simulink model "Skematik (Bismillah)"  (R2024b)
settings: Solver=ode23tb  StartTime=0.0  StopTime=10.0  RelTol=1e-3
undefined symbols (not defined in the file): D1, Delta
libraries: spsThreePhaseBreakerLib x78, spsThreePhaseParallelRLCLoadLib x39, spsThreePhasePISectionLineLib x26, spsThreePhaseTransformerTwoWindingsLib x18, spsExcitationSystemLib x4, spsSynchronousMachinepuStandardLib x4, spsMultimeterLib x1, spspowerguiLib x1
settings Model: Creator=Laika  LastModifiedBy=ACER
settings SolverCC: AlgebraicLoopSolver=TrustRegion
settings ModelReferenceCC: EnableRefExpFcnMdlSchedulingChecks=on
settings RTWCC: GPUComputeCapability=3.5  DLArmComputeVersion=19.05

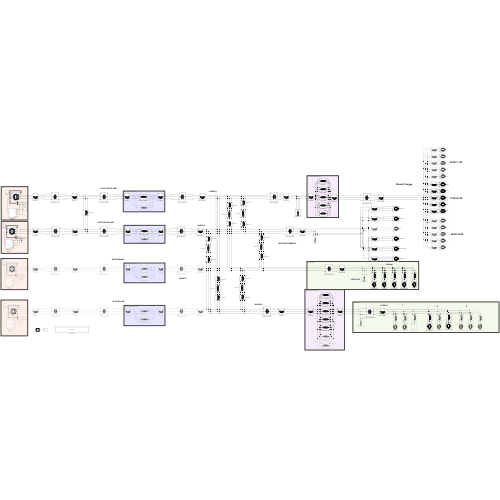
[thumbnail: Simulink's stored preview of the top-level diagram]
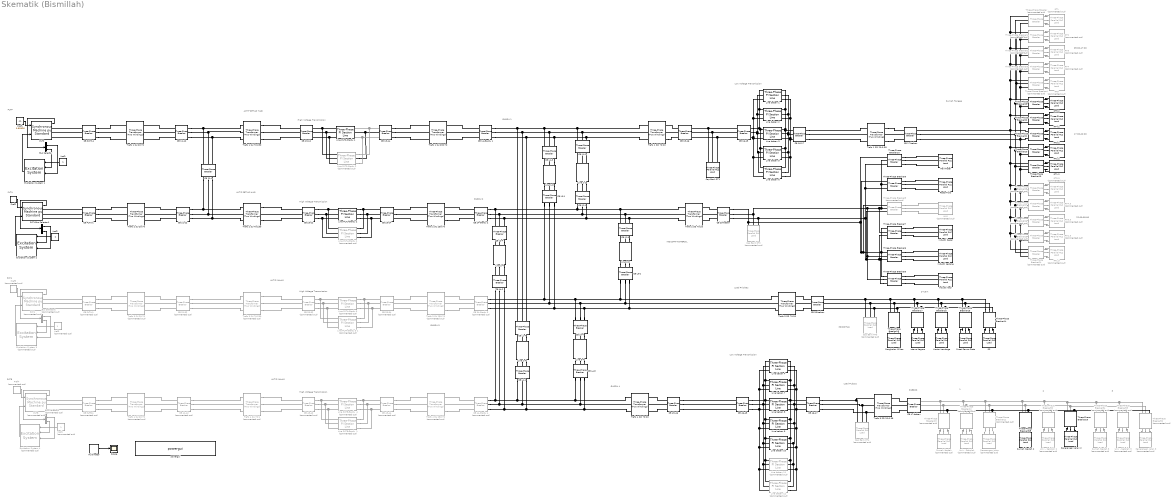
== system Skematik (Bismillah) ==
  note: High Voltage Transmission
  note: High Voltage Transmission
  note: High Voltage Transmission
  note: High Voltage Transmission
  note: Low Voltage Transmission
  note: Load Pubsos
  note: Load Prioritas
  note: Low Voltage Transmission
  note: PLTB
  note: PLTA
  note: PLTU
  note: PLTP
  note: GARDU 2
  note: GARDU 1
  note: GARDU 3
  note: GARDU 4
  note: AKTIF MALAM
  note: AKTIF MALAM
  note: AKTIF SETIAP HARI
  note: AKTIF SETIAP HARI
  note: INDUSTRI-KOMERSIL
  note: PRIORITAS
  note: PUBSOS
  note: 05:00-17:00
  note: 24 Jam
  note: 1
  note: 3
  note: 2
  note: 17:00-22:00
  note: 22:00-05:00
  note: Rumah Tangga
  Bus Selector : BusSelector  OutputSignals="dq0 components.Stator voltage  vq (pu),dq0 components.Stator voltage  vd (pu)"
  Bus Selector1 : BusSelector  OutputSignals="dq0 components.Stator voltage  vq (pu),dq0 components.Stator voltage  vd (pu)"
  Bus Selector2 : BusSelector  Commented=on  OutputSignals="dq0 components.Stator voltage  vq (pu),dq0 components.Stator voltage  vd (pu)"
  Bus Selector3 : BusSelector  Commented=on  OutputSignals="dq0 components.Stator voltage  vq (pu),dq0 components.Stator voltage  vd (pu)"
  CB 11-1 : spsThreePhaseBreakerLib/Three-Phase Breaker  InitialState=closed  SwitchA=off  SwitchB=off  SwitchC=off  SwitchTimes="[4/60  10/60]"  External=off  BreakerResistance=0.001  SnubberResistance=1e6  SnubberCapacitance=inf  Measurements=None
  CB 11-12 : spsThreePhaseBreakerLib/Three-Phase Breaker  InitialState=closed  SwitchA=off  SwitchB=off  SwitchC=off  SwitchTimes="[4/60  10/60]"  External=off  BreakerResistance=0.001  SnubberResistance=1e6  SnubberCapacitance=inf  Measurements=None
  CB 13-12 : spsThreePhaseBreakerLib/Three-Phase Breaker  InitialState=closed  SwitchA=off  SwitchB=off  SwitchC=off  SwitchTimes="[4/60  10/60]"  External=off  BreakerResistance=0.001  SnubberResistance=1e6  SnubberCapacitance=inf  Measurements=None
  CB 13-14 : spsThreePhaseBreakerLib/Three-Phase Breaker  InitialState=closed  SwitchA=off  SwitchB=off  SwitchC=off  SwitchTimes="[4/60  10/60]"  External=off  BreakerResistance=0.001  SnubberResistance=1e6  SnubberCapacitance=inf  Measurements=None
  CB 14-Gardu 1 : spsThreePhaseBreakerLib/Three-Phase Breaker  InitialState=closed  SwitchA=off  SwitchB=off  SwitchC=off  SwitchTimes="[4/60  10/60]"  External=off  BreakerResistance=0.001  SnubberResistance=1e6  SnubberCapacitance=inf  Measurements=None
  CB 15-16 : spsThreePhaseBreakerLib/Three-Phase Breaker  InitialState=closed  SwitchA=off  SwitchB=off  SwitchC=off  SwitchTimes="[4/60  10/60]"  External=off  BreakerResistance=0.001  SnubberResistance=1e6  SnubberCapacitance=inf  Measurements=None
  CB 16-15 : spsThreePhaseBreakerLib/Three-Phase Breaker  InitialState=closed  SwitchA=off  SwitchB=off  SwitchC=off  SwitchTimes="[4/60  10/60]"  External=off  BreakerResistance=0.001  SnubberResistance=1e6  SnubberCapacitance=inf  Measurements=None
  CB 16-17 : spsThreePhaseBreakerLib/Three-Phase Breaker  InitialState=closed  SwitchA=off  SwitchB=off  SwitchC=off  SwitchTimes="[4/60  10/60]"  External=off  BreakerResistance=0.001  SnubberResistance=1e6  SnubberCapacitance=inf  Measurements=None
  CB 17-beban : spsThreePhaseBreakerLib/Three-Phase Breaker  InitialState=closed  SwitchA=off  SwitchB=off  SwitchC=off  SwitchTimes="[4/60  10/60]"  External=off  BreakerResistance=1e-7  SnubberResistance=1e6  SnubberCapacitance=inf  Measurements=None
  CB 21-22 : spsThreePhaseBreakerLib/Three-Phase Breaker  InitialState=closed  SwitchA=off  SwitchB=off  SwitchC=off  SwitchTimes="[4/60  10/60]"  External=off  BreakerResistance=0.001  SnubberResistance=1e6  SnubberCapacitance=inf  Measurements=None
  CB 23-22 : spsThreePhaseBreakerLib/Three-Phase Breaker  InitialState=closed  SwitchA=off  SwitchB=off  SwitchC=off  SwitchTimes="[4/60  10/60]"  External=off  BreakerResistance=0.001  SnubberResistance=1e6  SnubberCapacitance=inf  Measurements=None
  CB 23-24 : spsThreePhaseBreakerLib/Three-Phase Breaker  InitialState=closed  SwitchA=off  SwitchB=off  SwitchC=off  SwitchTimes="[4/60  10/60]"  External=off  BreakerResistance=0.001  SnubberResistance=1e6  SnubberCapacitance=inf  Measurements=None
  CB 24-Gardu 2 : spsThreePhaseBreakerLib/Three-Phase Breaker  InitialState=closed  SwitchA=off  SwitchB=off  SwitchC=off  SwitchTimes="[4/60  10/60]"  External=off  BreakerResistance=0.001  SnubberResistance=1e6  SnubberCapacitance=inf  Measurements=None
  CB 25-beban : spsThreePhaseBreakerLib/Three-Phase Breaker  InitialState=closed  SwitchA=off  SwitchB=off  SwitchC=off  SwitchTimes="[4/60  10/60]"  External=off  BreakerResistance=1e-7  SnubberResistance=1e6  SnubberCapacitance=inf  Measurements=None
  CB 31-32 : spsThreePhaseBreakerLib/Three-Phase Breaker  Commented=on  InitialState=closed  SwitchA=off  SwitchB=off  SwitchC=off  SwitchTimes="[4/60  10/60]"  External=off  BreakerResistance=0.001  SnubberResistance=1e6  SnubberCapacitance=inf  Measurements=None
  CB 33-32 : spsThreePhaseBreakerLib/Three-Phase Breaker  Commented=on  InitialState=closed  SwitchA=off  SwitchB=off  SwitchC=off  SwitchTimes="[4/60  10/60]"  External=off  BreakerResistance=0.001  SnubberResistance=1e6  SnubberCapacitance=inf  Measurements=None
  CB 33-34 : spsThreePhaseBreakerLib/Three-Phase Breaker  Commented=on  InitialState=closed  SwitchA=off  SwitchB=off  SwitchC=off  SwitchTimes="[4/60  10/60]"  External=off  BreakerResistance=0.001  SnubberResistance=1e6  SnubberCapacitance=inf  Measurements=None
  CB 34-Gardu 3 : spsThreePhaseBreakerLib/Three-Phase Breaker  Commented=on  InitialState=closed  SwitchA=off  SwitchB=off  SwitchC=off  SwitchTimes="[4/60  10/60]"  External=off  BreakerResistance=0.001  SnubberResistance=1e6  SnubberCapacitance=inf  Measurements=None
  CB 35-beban : spsThreePhaseBreakerLib/Three-Phase Breaker  InitialState=closed  SwitchA=off  SwitchB=off  SwitchC=off  SwitchTimes="[4/60  10/60]"  External=off  BreakerResistance=1e-7  SnubberResistance=1e6  SnubberCapacitance=inf  Measurements=None
  CB 41-42 : spsThreePhaseBreakerLib/Three-Phase Breaker  Commented=on  InitialState=closed  SwitchA=off  SwitchB=off  SwitchC=off  SwitchTimes="[4/60  10/60]"  External=off  BreakerResistance=0.001  SnubberResistance=1e6  SnubberCapacitance=inf  Measurements=None
  CB 43-42 : spsThreePhaseBreakerLib/Three-Phase Breaker  Commented=on  InitialState=closed  SwitchA=off  SwitchB=off  SwitchC=off  SwitchTimes="[4/60  10/60]"  External=off  BreakerResistance=0.001  SnubberResistance=1e6  SnubberCapacitance=inf  Measurements=None
  CB 43-44 : spsThreePhaseBreakerLib/Three-Phase Breaker  Commented=on  InitialState=closed  SwitchA=off  SwitchB=off  SwitchC=off  SwitchTimes="[4/60  10/60]"  External=off  BreakerResistance=0.001  SnubberResistance=1e6  SnubberCapacitance=inf  Measurements=None
  CB 44-Gardu 4 : spsThreePhaseBreakerLib/Three-Phase Breaker  Commented=on  InitialState=closed  SwitchA=off  SwitchB=off  SwitchC=off  SwitchTimes="[4/60  10/60]"  External=off  BreakerResistance=0.001  SnubberResistance=1e6  SnubberCapacitance=inf  Measurements=None
  CB 45-46 : spsThreePhaseBreakerLib/Three-Phase Breaker  InitialState=closed  SwitchA=off  SwitchB=off  SwitchC=off  SwitchTimes="[4/60  10/60]"  External=off  BreakerResistance=0.001  SnubberResistance=1e6  SnubberCapacitance=inf  Measurements=None
  CB 46-45 : spsThreePhaseBreakerLib/Three-Phase Breaker  InitialState=closed  SwitchA=off  SwitchB=off  SwitchC=off  SwitchTimes="[4/60  10/60]"  External=off  BreakerResistance=0.001  SnubberResistance=1e6  SnubberCapacitance=inf  Measurements=None
  CB 46-47 : spsThreePhaseBreakerLib/Three-Phase Breaker  InitialState=closed  SwitchA=off  SwitchB=off  SwitchC=off  SwitchTimes="[4/60  10/60]"  External=off  BreakerResistance=0.001  SnubberResistance=1e6  SnubberCapacitance=inf  Measurements=None
  CB 47-beban : spsThreePhaseBreakerLib/Three-Phase Breaker  InitialState=closed  SwitchA=off  SwitchB=off  SwitchC=off  SwitchTimes="[4/60  10/60]"  External=off  BreakerResistance=1e-7  SnubberResistance=1e6  SnubberCapacitance=inf  Measurements=None
  CB L1-2 : spsThreePhaseBreakerLib/Three-Phase Breaker  InitialState=closed  SwitchA=off  SwitchB=off  SwitchC=off  SwitchTimes="[4/60  10/60]"  External=off  BreakerResistance=0.001  SnubberResistance=1e6  SnubberCapacitance=inf  Measurements=None
  CB L1-3 : spsThreePhaseBreakerLib/Three-Phase Breaker  InitialState=closed  SwitchA=off  SwitchB=off  SwitchC=off  SwitchTimes="[4/60  10/60]"  External=off  BreakerResistance=0.001  SnubberResistance=1e6  SnubberCapacitance=inf  Measurements=None
  CB L1-4 : spsThreePhaseBreakerLib/Three-Phase Breaker  InitialState=closed  SwitchA=off  SwitchB=off  SwitchC=off  SwitchTimes="[4/60  10/60]"  External=off  BreakerResistance=0.001  SnubberResistance=1e6  SnubberCapacitance=inf  Measurements=None
  CB L2-1 : spsThreePhaseBreakerLib/Three-Phase Breaker  InitialState=closed  SwitchA=off  SwitchB=off  SwitchC=off  SwitchTimes="[4/60  10/60]"  External=off  BreakerResistance=0.001  SnubberResistance=1e6  SnubberCapacitance=inf  Measurements=None
  CB L2-3 : spsThreePhaseBreakerLib/Three-Phase Breaker  InitialState=closed  SwitchA=off  SwitchB=off  SwitchC=off  SwitchTimes="[4/60  10/60]"  External=off  BreakerResistance=0.001  SnubberResistance=1e6  SnubberCapacitance=inf  Measurements=None
  CB L2-4 : spsThreePhaseBreakerLib/Three-Phase Breaker  InitialState=closed  SwitchA=off  SwitchB=off  SwitchC=off  SwitchTimes="[4/60  10/60]"  External=off  BreakerResistance=0.001  SnubberResistance=1e6  SnubberCapacitance=inf  Measurements=None
  CB L3-1 : spsThreePhaseBreakerLib/Three-Phase Breaker  InitialState=closed  SwitchA=off  SwitchB=off  SwitchC=off  SwitchTimes="[4/60  10/60]"  External=off  BreakerResistance=0.001  SnubberResistance=1e6  SnubberCapacitance=inf  Measurements=None
  CB L3-2 : spsThreePhaseBreakerLib/Three-Phase Breaker  InitialState=closed  SwitchA=off  SwitchB=off  SwitchC=off  SwitchTimes="[4/60  10/60]"  External=off  BreakerResistance=0.001  SnubberResistance=1e6  SnubberCapacitance=inf  Measurements=None
  CB L3-4 : spsThreePhaseBreakerLib/Three-Phase Breaker  InitialState=closed  SwitchA=off  SwitchB=off  SwitchC=off  SwitchTimes="[4/60  10/60]"  External=off  BreakerResistance=0.001  SnubberResistance=1e6  SnubberCapacitance=inf  Measurements=None
  CB L4-1 : spsThreePhaseBreakerLib/Three-Phase Breaker  InitialState=closed  SwitchA=off  SwitchB=off  SwitchC=off  SwitchTimes="[4/60  10/60]"  External=off  BreakerResistance=0.001  SnubberResistance=1e6  SnubberCapacitance=inf  Measurements=None
  CB L4-2 : spsThreePhaseBreakerLib/Three-Phase Breaker  InitialState=closed  SwitchA=off  SwitchB=off  SwitchC=off  SwitchTimes="[4/60  10/60]"  External=off  BreakerResistance=0.001  SnubberResistance=1e6  SnubberCapacitance=inf  Measurements=None
  CB L4-3 : spsThreePhaseBreakerLib/Three-Phase Breaker  InitialState=closed  SwitchA=off  SwitchB=off  SwitchC=off  SwitchTimes="[4/60  10/60]"  External=off  BreakerResistance=0.001  SnubberResistance=1e6  SnubberCapacitance=inf  Measurements=None
  CB PLTA-1 : spsThreePhaseBreakerLib/Three-Phase Breaker  Commented=on  InitialState=closed  SwitchA=off  SwitchB=off  SwitchC=off  SwitchTimes="[4/60  10/60]"  External=off  BreakerResistance=0.001  SnubberResistance=1e6  SnubberCapacitance=inf  Measurements=None
  CB PLTB-1 : spsThreePhaseBreakerLib/Three-Phase Breaker  Commented=on  InitialState=closed  SwitchA=off  SwitchB=off  SwitchC=off  SwitchTimes="[4/60  10/60]"  External=off  BreakerResistance=0.001  SnubberResistance=1e6  SnubberCapacitance=inf  Measurements=None
  CB PLTP-1 : spsThreePhaseBreakerLib/Three-Phase Breaker  InitialState=closed  SwitchA=off  SwitchB=off  SwitchC=off  SwitchTimes="[4/60  10/60]"  External=off  BreakerResistance=0.001  SnubberResistance=1e6  SnubberCapacitance=inf  Measurements=None
  CB PLTU-1 : spsThreePhaseBreakerLib/Three-Phase Breaker  InitialState=closed  SwitchA=off  SwitchB=off  SwitchC=off  SwitchTimes="[4/60  10/60]"  External=off  BreakerResistance=0.001  SnubberResistance=1e6  SnubberCapacitance=inf  Measurements=None
  Cap Bank RT1 : spsThreePhaseParallelRLCLoadLib/Three-Phase Parallel RLC Load  LConnTagsString=A|B|C  Configuration=Y (grounded)  NominalVoltage=20e3  Vabc=[1e3 1e3 1e3]  Vabcp=[1e3 1e3 1e3]  NominalFrequency=50  UnbalancedPower=off  ActivePower=0  InductivePower=0  CapacitivePower=60e6  Pabc=[10e3 9e3 11e3]  QLabc=[100 90 110]  QCabc=[100 90 110]  Pabcp=[10e3 9e3 11e3]  QLabcp=[100 90 110]  QCabcp=[100 90 110]  Measurements=Branch voltages and currents  LoadType=constant Z
  Cap Bank RT2 : spsThreePhaseParallelRLCLoadLib/Three-Phase Parallel RLC Load  Commented=on  LConnTagsString=A|B|C  Configuration=Y (grounded)  NominalVoltage=20e3  Vabc=[1e3 1e3 1e3]  Vabcp=[1e3 1e3 1e3]  NominalFrequency=50  UnbalancedPower=off  ActivePower=0  InductivePower=0  CapacitivePower=50e3  Pabc=[10e3 9e3 11e3]  QLabc=[100 90 110]  QCabc=[100 90 110]  Pabcp=[10e3 9e3 11e3]  QLabcp=[100 90 110]  QCabcp=[100 90 110]  Measurements=Branch voltages and currents  LoadType=constant Z
  Cap Bank RT3 : spsThreePhaseParallelRLCLoadLib/Three-Phase Parallel RLC Load  Commented=on  LConnTagsString=A|B|C  Configuration=Y (grounded)  NominalVoltage=20e3  Vabc=[1e3 1e3 1e3]  Vabcp=[1e3 1e3 1e3]  NominalFrequency=50  UnbalancedPower=off  ActivePower=0  InductivePower=0  CapacitivePower=50e3  Pabc=[10e3 9e3 11e3]  QLabc=[100 90 110]  QCabc=[100 90 110]  Pabcp=[10e3 9e3 11e3]  QLabcp=[100 90 110]  QCabcp=[100 90 110]  Measurements=Branch voltages and currents  LoadType=constant Z
  Cap Bank RT4 : spsThreePhaseParallelRLCLoadLib/Three-Phase Parallel RLC Load  Commented=on  LConnTagsString=A|B|C  Configuration=Y (grounded)  NominalVoltage=20e3  Vabc=[1e3 1e3 1e3]  Vabcp=[1e3 1e3 1e3]  NominalFrequency=50  UnbalancedPower=off  ActivePower=0  InductivePower=0  CapacitivePower=0.75e6  Pabc=[10e3 9e3 11e3]  QLabc=[100 90 110]  QCabc=[100 90 110]  Pabcp=[10e3 9e3 11e3]  QLabcp=[100 90 110]  QCabcp=[100 90 110]  Measurements=Branch voltages and currents  LoadType=constant Z
  Excitation System 1 : spsExcitationSystemLib/Excitation System  tr=20e-3  reg=[ 300, 0.001 ]  exc=[ 1, 0 ]  tgr=[ 0, 0 ]  damp=[ 0.001, 0.1 ]  sat=[ 0, 0 ]  lim=[ -11.5, 11.5, 0 ]  v0=[1 18.415]
  Excitation System 2 : spsExcitationSystemLib/Excitation System  tr=20e-3  reg=[ 300, 0.001 ]  exc=[ 1, 0 ]  tgr=[ 0, 0 ]  damp=[ 0.001, 0.1 ]  sat=[ 0, 0 ]  lim=[ -11.5, 11.5, 0 ]  v0=[1 13.043]
  Excitation System 3 : spsExcitationSystemLib/Excitation System  Commented=on  tr=20e-3  reg=[ 300, 0.001 ]  exc=[ 1, 0 ]  tgr=[ 0, 0 ]  damp=[ 0.001, 0.1 ]  sat=[ 0, 0 ]  lim=[ -11.5, 11.5, 0 ]  v0=[1 2.1735]
  Excitation System 4 : spsExcitationSystemLib/Excitation System  Commented=on  tr=20e-3  reg=[ 300, 0.001 ]  exc=[ 1, 0 ]  tgr=[ 0, 0 ]  damp=[ 0.001, 0.1 ]  sat=[ 0, 0 ]  lim=[ -11.5, 11.5, 0 ]  v0=[1 12.474]
  Industri besar : spsThreePhaseParallelRLCLoadLib/Three-Phase Parallel RLC Load  LConnTagsString=A|B|C  Configuration=Y (grounded)  NominalVoltage=20e3  Vabc=[1e3 1e3 1e3]  Vabcp=[1e3 1e3 1e3]  NominalFrequency=50  UnbalancedPower=off  ActivePower=9e5  InductivePower=4.36e5  CapacitivePower=0  Pabc=[10e3 9e3 11e3]  QLabc=[100 90 110]  QCabc=[100 90 110]  Pabcp=[10e3 9e3 11e3]  QLabcp=[100 90 110]  QCabcp=[100 90 110]  Measurements=Branch voltages and currents  LoadType=constant Z
  Industri kecil : spsThreePhaseParallelRLCLoadLib/Three-Phase Parallel RLC Load  LConnTagsString=A|B|C  Configuration=Y (grounded)  NominalVoltage=20e3  Vabc=[1e3 1e3 1e3]  Vabcp=[1e3 1e3 1e3]  NominalFrequency=50  UnbalancedPower=off  ActivePower=5.94e5  InductivePower=2.88e5  CapacitivePower=0  Pabc=[10e3 9e3 11e3]  QLabc=[100 90 110]  QCabc=[100 90 110]  Pabcp=[10e3 9e3 11e3]  QLabcp=[100 90 110]  QCabcp=[100 90 110]  Measurements=Branch voltages and currents  LoadType=constant Z
  Industri sedang : spsThreePhaseParallelRLCLoadLib/Three-Phase Parallel RLC Load  LConnTagsString=A|B|C  Configuration=Y (grounded)  NominalVoltage=20e3  Vabc=[1e3 1e3 1e3]  Vabcp=[1e3 1e3 1e3]  NominalFrequency=50  UnbalancedPower=off  ActivePower=4.5e6  InductivePower=2.18e6  CapacitivePower=0  Pabc=[10e3 9e3 11e3]  QLabc=[100 90 110]  QCabc=[100 90 110]  Pabcp=[10e3 9e3 11e3]  QLabcp=[100 90 110]  QCabcp=[100 90 110]  Measurements=Branch voltages and currents  LoadType=constant Z
  Istana Negara : spsThreePhaseParallelRLCLoadLib/Three-Phase Parallel RLC Load  LConnTagsString=A|B|C  Configuration=Y (grounded)  NominalVoltage=20e3  Vabc=[1e3 1e3 1e3]  Vabcp=[1e3 1e3 1e3]  NominalFrequency=50  UnbalancedPower=off  ActivePower=9e4  InductivePower=4.36e4  CapacitivePower=0  Pabc=[10e3 9e3 11e3]  QLabc=[100 90 110]  QCabc=[100 90 110]  Pabcp=[10e3 9e3 11e3]  QLabcp=[100 90 110]  QCabcp=[100 90 110]  Measurements=Branch voltages and currents  LoadType=constant Z
  Kantor Lembaga : spsThreePhaseParallelRLCLoadLib/Three-Phase Parallel RLC Load  LConnTagsString=A|B|C  Configuration=Y (grounded)  NominalVoltage=20e3  Vabc=[1e3 1e3 1e3]  Vabcp=[1e3 1e3 1e3]  NominalFrequency=50  UnbalancedPower=off  ActivePower=9e4  InductivePower=4.36e4  CapacitivePower=0  Pabc=[10e3 9e3 11e3]  QLabc=[100 90 110]  QCabc=[100 90 110]  Pabcp=[10e3 9e3 11e3]  QLabcp=[100 90 110]  QCabcp=[100 90 110]  Measurements=Branch voltages and currents  LoadType=constant Z
  Line 1-1 : spsThreePhasePISectionLineLib/Three-Phase PI Section Line  LConnTagsString=a|b|c  RConnTagsString=A|B|C  Length=20  Frequency=50  Resistances=[ 0.002 0.3864]  Inductances="[ 6.3694e-3  4.1264e-3]"  Capacitances=[12.74e-9 7.751e-9]
  Line 1-3 : spsThreePhasePISectionLineLib/Three-Phase PI Section Line  LConnTagsString=a|b|c  RConnTagsString=A|B|C  Length=5  Frequency=50  Resistances=[ 0.002 0.3864]  Inductances="[ 6.3694e-3  4.1264e-3]"  Capacitances=[12.74e-9 7.751e-9]
  Line 1-4 : spsThreePhasePISectionLineLib/Three-Phase PI Section Line  LConnTagsString=a|b|c  RConnTagsString=A|B|C  Length=20  Frequency=50  Resistances=[ 0.002 0.3864]  Inductances="[ 6.3694e-3  4.1264e-3]"  Capacitances=[12.74e-9 7.751e-9]
  Line 2-3 : spsThreePhasePISectionLineLib/Three-Phase PI Section Line  LConnTagsString=a|b|c  RConnTagsString=A|B|C  Length=5  Frequency=50  Resistances=[ 0.002 0.3864]  Inductances="[ 6.3694e-3  4.1264e-3]"  Capacitances=[12.74e-9 7.751e-9]
  Line 2-4 : spsThreePhasePISectionLineLib/Three-Phase PI Section Line  LConnTagsString=a|b|c  RConnTagsString=A|B|C  Length=20  Frequency=50  Resistances=[ 0.002 0.3864]  Inductances="[ 6.3694e-3  4.1264e-3]"  Capacitances=[12.74e-9 7.751e-9]
  Line 3-4 : spsThreePhasePISectionLineLib/Three-Phase PI Section Line  LConnTagsString=a|b|c  RConnTagsString=A|B|C  Length=5  Frequency=50  Resistances=[ 0.002 0.3864]  Inductances="[ 6.3694e-3  4.1264e-3]"  Capacitances=[12.74e-9 7.751e-9]
  "Line PLTA-Gardu 3 " : spsThreePhasePISectionLineLib/Three-Phase PI Section Line  Commented=on  LConnTagsString=a|b|c  RConnTagsString=A|B|C  Length=50  Frequency=50  Resistances=[ 0.002 0.3864]  Inductances="[ 6.3694e-3  4.1264e-3]"  Capacitances=[12.74e-9 7.751e-9]
  Line PLTA-Gardu 3 1 : spsThreePhasePISectionLineLib/Three-Phase PI Section Line  Commented=on  LConnTagsString=a|b|c  RConnTagsString=A|B|C  Length=50  Frequency=50  Resistances=[ 0.002 0.3864]  Inductances="[ 6.3694e-3  4.1264e-3]"  Capacitances=[12.74e-9 7.751e-9]
  Line PLTB-Gardu  1 : spsThreePhasePISectionLineLib/Three-Phase PI Section Line  Commented=on  LConnTagsString=a|b|c  RConnTagsString=A|B|C  Length=20  Frequency=50  Resistances=[ 0.002 0.3864]  Inductances="[ 6.3694e-3  4.1264e-3]"  Capacitances=[12.74e-9 7.751e-9]
  Line PLTB-Gardu  4 : spsThreePhasePISectionLineLib/Three-Phase PI Section Line  Commented=on  LConnTagsString=a|b|c  RConnTagsString=A|B|C  Length=20  Frequency=50  Resistances=[ 0.002 0.3864]  Inductances="[ 6.3694e-3  4.1264e-3]"  Capacitances=[12.74e-9 7.751e-9]
  Line PLTP-Gardu 1 : spsThreePhasePISectionLineLib/Three-Phase PI Section Line  LConnTagsString=a|b|c  RConnTagsString=A|B|C  Length=100  Frequency=50  Resistances=[ 0.002 0.3864]  Inductances="[ 6.3694e-3  4.1264e-3]"  Capacitances=[12.74e-9 7.751e-9]
  Line PLTP-Gardu 2 : spsThreePhasePISectionLineLib/Three-Phase PI Section Line  Commented=on  LConnTagsString=a|b|c  RConnTagsString=A|B|C  Length=100  Frequency=50  Resistances=[ 0.002 0.3864]  Inductances="[ 6.3694e-3  4.1264e-3]"  Capacitances=[12.74e-9 7.751e-9]
  Line PLTU-Gardu 1 : spsThreePhasePISectionLineLib/Three-Phase PI Section Line  Commented=on  LConnTagsString=a|b|c  RConnTagsString=A|B|C  Length=100  Frequency=50  Resistances=[ 0.002 0.3864]  Inductances="[ 6.3694e-3  4.1264e-3]"  Capacitances=[12.74e-9 7.751e-9]
  Line PLTU-Gardu 2 : spsThreePhasePISectionLineLib/Three-Phase PI Section Line  LConnTagsString=a|b|c  RConnTagsString=A|B|C  Length=100  Frequency=50  Resistances=[ 0.002 0.3864]  Inductances="[ 6.3694e-3  4.1264e-3]"  Capacitances=[12.74e-9 7.751e-9]
  Line beban {1..10} (10 alike) : spsThreePhasePISectionLineLib/Three-Phase PI Section Line  LConnTagsString=a|b|c  RConnTagsString=A|B|C  Length=3  Frequency=50  Resistances=[ 0.002 0.3864]  Inductances="[ 6.3694e-3  4.1264e-3]"  Capacitances=[12.74e-9 7.751e-9]
  Line beban 11 : spsThreePhasePISectionLineLib/Three-Phase PI Section Line  Commented=on  LConnTagsString=a|b|c  RConnTagsString=A|B|C  Length=3  Frequency=50  Resistances=[ 0.002 0.3864]  Inductances="[ 6.3694e-3  4.1264e-3]"  Capacitances=[12.74e-9 7.751e-9]
  Line beban 12 : spsThreePhasePISectionLineLib/Three-Phase PI Section Line  Commented=on  LConnTagsString=a|b|c  RConnTagsString=A|B|C  Length=3  Frequency=50  Resistances=[ 0.002 0.3864]  Inductances="[ 6.3694e-3  4.1264e-3]"  Capacitances=[12.74e-9 7.751e-9]
  Mall-Hotel : spsThreePhaseParallelRLCLoadLib/Three-Phase Parallel RLC Load  LConnTagsString=A|B|C  Configuration=Y (grounded)  NominalVoltage=20e3  Vabc=[1e3 1e3 1e3]  Vabcp=[1e3 1e3 1e3]  NominalFrequency=50  UnbalancedPower=off  ActivePower=9e4  InductivePower=4.36e4  CapacitivePower=0  Pabc=[10e3 9e3 11e3]  QLabc=[100 90 110]  QCabc=[100 90 110]  Pabcp=[10e3 9e3 11e3]  QLabcp=[100 90 110]  QCabcp=[100 90 110]  Measurements=Branch voltages and currents  LoadType=constant Z
  Multimeter : spsMultimeterLib/Multimeter  L=216  sel=[7 8 9 10 11 12 13 14 15 16 17 18 19 20 21 22 23 24 25 26 27 34 35 36 37 38 39 67 68 69 76 77 78 85 86 87 97 98 99]  yselected={}  Gain=[1 1 1 1 1 1 1 1 1 1 1 1 1 1 1 1 1 1 1 1 1 1 1 1 1 1 1 1 1 1 1 1 1 1 1 1 1 1 1]  OutputType=Magnitude  PlotAtSimulationStop=off  PhasorSimulation=off
  PLTA : spsSynchronousMachinepuStandardLib/Synchronous Machine pu Standard  Commented=on  PresetModel=No  MechanicalLoad=Mechanical power Pm  ShowDetailedParameters=on  RotorType=Salient-pole  Units=per unit standard parameters  MeasurementBus=off  NominalParameters="[ 30e6/0.95  20e3   50]"  Reactances1=[ 1.81, 0.3, 0.23, 1.76, 0.65, 0.25, 0.15 ]  Reactances2="[ 1.305, 0.296, 0.252, 0.474,  0.243,  0.1 ]"  dAxisTimeConstants=Open-circuit  qAxisTimeConstants=Short-circuit  TimeConstants1="[ 4.4849  0.0681  0.1  ]"  TimeConstants2=[ 8.0, 0.03, 1.0, 0.07 ]  TimeConstants3="[  4.49  0.0681  0.0513  ]"  TimeConstants4=[ 8.0, 0.03, 0.3371, 0.0295 ]  TimeConstants5=[ 1.01, 0.053, 0.1 ]  TimeConstants6=[ 1.3201, 0.023, 1.0, 0.07 ]  TimeConstants7=[0.012 0.003 0.003]  TimeConstants8=[ 1.3201, 0.0231, 0.3371, 0.0295 ]  StatorResistance=0.003  Mechanical=[ 3.7 0 20 ]  PolePairs=20  InitialConditions=[0 -124.504 1.57718 1.57718 1.57718 -173.405 -293.405 -53.4047 2.17353]  SetSaturation=off  Saturation=[0.6404,0.7127,0.8441,0.9214,0.9956,1.082,1.19,1.316,1.457;0.7,0.7698,0.8872,0.9466,0.9969,1.046,1.1,1.151,1.201]  LoadFlowParameters=[1 120000000 0 0 0]  TsPowergui=0  TsBlock=-1  IterativeModel=Forward Euler  IterativeDiscreteModel=Trapezoidal non iterative  BusType=swing  Pref=100000000  Qref=0  Qmin=-Inf  Qmax=Inf  PLF=0  QLF=0
  PLTB : spsSynchronousMachinepuStandardLib/Synchronous Machine pu Standard  Commented=on  PresetModel=No  MechanicalLoad=Mechanical power Pm  ShowDetailedParameters=on  RotorType=Salient-pole  Units=per unit standard parameters  MeasurementBus=off  NominalParameters="[ 10e6/0.96  20e3   50]"  Reactances1=[ 1.81, 0.3, 0.23, 1.76, 0.65, 0.25, 0.15 ]  Reactances2="[ 1.305, 0.296, 0.252, 0.474,  0.243,  0.1 ]"  dAxisTimeConstants=Open-circuit  qAxisTimeConstants=Short-circuit  TimeConstants1="[ 4.4849  0.0681  0.1  ]"  TimeConstants2=[ 8.0, 0.03, 1.0, 0.07 ]  TimeConstants3="[  4.49  0.0681  0.0513  ]"  TimeConstants4=[ 8.0, 0.03, 0.3371, 0.0295 ]  TimeConstants5=[ 1.01, 0.053, 0.1 ]  TimeConstants6=[ 1.3201, 0.023, 1.0, 0.07 ]  TimeConstants7=[0.012 0.003 0.003]  TimeConstants8=[ 1.3201, 0.0231, 0.3371, 0.0295 ]  StatorResistance=0.003  Mechanical=[ 3.7 0 20 ]  PolePairs=20  InitialConditions=[0 -1.70334 9.60252 9.60252 9.60252 10.9686 -109.031 130.969 12.474]  SetSaturation=off  Saturation=[0.6404,0.7127,0.8441,0.9214,0.9956,1.082,1.19,1.316,1.457;0.7,0.7698,0.8872,0.9466,0.9969,1.046,1.1,1.151,1.201]  LoadFlowParameters=[1 120000000 0 0 0]  TsPowergui=0  TsBlock=-1  IterativeModel=Forward Euler  IterativeDiscreteModel=Trapezoidal non iterative  BusType=PV  Pref=100000000  Qref=0  Qmin=-Inf  Qmax=Inf  PLF=0  QLF=0
  PLTP : spsSynchronousMachinepuStandardLib/Synchronous Machine pu Standard  PresetModel=No  MechanicalLoad=Mechanical power Pm  ShowDetailedParameters=on  RotorType=Salient-pole  Units=per unit standard parameters  MeasurementBus=off  NominalParameters="[ 80e6/0.9  20e3   50]"  Reactances1=[ 1.81, 0.3, 0.23, 1.76, 0.65, 0.25, 0.15 ]  Reactances2="[ 1.305, 0.296, 0.252, 0.474,  0.243,  0.1 ]"  dAxisTimeConstants=Open-circuit  qAxisTimeConstants=Short-circuit  TimeConstants1="[ 4.4849  0.0681  0.1  ]"  TimeConstants2=[ 8.0, 0.03, 1.0, 0.07 ]  TimeConstants3="[  4.49  0.0681  0.0513  ]"  TimeConstants4=[ 8.0, 0.03, 0.3371, 0.0295 ]  TimeConstants5=[ 1.01, 0.053, 0.1 ]  TimeConstants6=[ 1.3201, 0.023, 1.0, 0.07 ]  TimeConstants7=[0.012 0.003 0.003]  TimeConstants8=[ 1.3201, 0.0231, 0.3371, 0.0295 ]  StatorResistance=0.003  Mechanical=[ 3.7 0 20 ]  PolePairs=20  InitialConditions=[0 -89.1081 13.3449 13.3449 13.3449 -88.6045 -208.604 31.3955 18.4147]  SetSaturation=off  Saturation=[0.6404,0.7127,0.8441,0.9214,0.9956,1.082,1.19,1.316,1.457;0.7,0.7698,0.8872,0.9466,0.9969,1.046,1.1,1.151,1.201]  LoadFlowParameters=[2 0 0 0 0]  TsPowergui=0  TsBlock=-1  IterativeModel=Forward Euler  IterativeDiscreteModel=Trapezoidal non iterative  BusType=swing  Pref=0  Qref=0  Qmin=-Inf  Qmax=Inf  PLF=0  QLF=0
  PLTU : spsSynchronousMachinepuStandardLib/Synchronous Machine pu Standard  PresetModel=No  MechanicalLoad=Mechanical power Pm  ShowDetailedParameters=on  RotorType=Salient-pole  Units=per unit standard parameters  MeasurementBus=off  NominalParameters="[ 100e6/0.9  20e3   50]"  Reactances1=[ 1.81, 0.3, 0.23, 1.76, 0.65, 0.25, 0.15 ]  Reactances2="[ 1.305, 0.296, 0.252, 0.474,  0.243,  0.1 ]"  dAxisTimeConstants=Open-circuit  qAxisTimeConstants=Short-circuit  TimeConstants1="[ 4.4849  0.0681  0.1  ]"  TimeConstants2=[ 8.0, 0.03, 1.0, 0.07 ]  TimeConstants3="[  4.49  0.0681  0.0513  ]"  TimeConstants4=[ 8.0, 0.03, 0.3371, 0.0295 ]  TimeConstants5=[ 1.01, 0.053, 0.1 ]  TimeConstants6=[ 1.3201, 0.023, 1.0, 0.07 ]  TimeConstants7=[0.012 0.003 0.003]  TimeConstants8=[ 1.3201, 0.0231, 0.3371, 0.0295 ]  StatorResistance=0.003  Mechanical=[ 3.7 0 20 ]  PolePairs=20  InitialConditions=[0 89.4306 10.7601 10.7601 10.7601 91.0487 -28.9513 211.049 13.0435]  SetSaturation=off  Saturation=[0.6404,0.7127,0.8441,0.9214,0.9956,1.082,1.19,1.316,1.457;0.7,0.7698,0.8872,0.9466,0.9969,1.046,1.1,1.151,1.201]  LoadFlowParameters=[1 120000000 0 0 0]  TsPowergui=0  TsBlock=-1  IterativeModel=Forward Euler  IterativeDiscreteModel=Trapezoidal non iterative  BusType=PV  Pref=100000000  Qref=0  Qmin=-Inf  Qmax=Inf  PLF=0  QLF=0
  Pangkalan Militer : spsThreePhaseParallelRLCLoadLib/Three-Phase Parallel RLC Load  LConnTagsString=A|B|C  Configuration=Y (grounded)  NominalVoltage=20e3  Vabc=[1e3 1e3 1e3]  Vabcp=[1e3 1e3 1e3]  NominalFrequency=50  UnbalancedPower=off  ActivePower=2.03e5  InductivePower=9.81e4  CapacitivePower=0  Pabc=[10e3 9e3 11e3]  QLabc=[100 90 110]  QCabc=[100 90 110]  Pabcp=[10e3 9e3 11e3]  QLabcp=[100 90 110]  QCabcp=[100 90 110]  Measurements=Branch voltages and currents  LoadType=constant Z
  Penerangan Jalan : spsThreePhaseParallelRLCLoadLib/Three-Phase Parallel RLC Load  Commented=on  LConnTagsString=A|B|C  Configuration=Y (grounded)  NominalVoltage=380  Vabc=[1e3 1e3 1e3]  Vabcp=[1e3 1e3 1e3]  NominalFrequency=50  UnbalancedPower=off  ActivePower=0  InductivePower=0  CapacitivePower=0  Pabc=[10e3 9e3 11e3]  QLabc=[100 90 110]  QCabc=[100 90 110]  Pabcp=[10e3 9e3 11e3]  QLabcp=[100 90 110]  QCabcp=[100 90 110]  Measurements=Branch voltages and currents  LoadType=constant Z
  Penerangan Jalan 2 : spsThreePhaseParallelRLCLoadLib/Three-Phase Parallel RLC Load  LConnTagsString=A|B|C  Configuration=Y (grounded)  NominalVoltage=380  Vabc=[1e3 1e3 1e3]  Vabcp=[1e3 1e3 1e3]  NominalFrequency=50  UnbalancedPower=off  ActivePower=1.8e5  InductivePower=8.72e4  CapacitivePower=0  Pabc=[10e3 9e3 11e3]  QLabc=[100 90 110]  QCabc=[100 90 110]  Pabcp=[10e3 9e3 11e3]  QLabcp=[100 90 110]  QCabcp=[100 90 110]  Measurements=Branch voltages and currents  LoadType=constant Z
  Penerangan Jalan 3 : spsThreePhaseParallelRLCLoadLib/Three-Phase Parallel RLC Load  Commented=on  LConnTagsString=A|B|C  Configuration=Y (grounded)  NominalVoltage=380  Vabc=[1e3 1e3 1e3]  Vabcp=[1e3 1e3 1e3]  NominalFrequency=50  UnbalancedPower=off  ActivePower=1.92e6  InductivePower=0.56e6  CapacitivePower=0  Pabc=[10e3 9e3 11e3]  QLabc=[100 90 110]  QCabc=[100 90 110]  Pabcp=[10e3 9e3 11e3]  QLabcp=[100 90 110]  QCabcp=[100 90 110]  Measurements=Branch voltages and currents  LoadType=constant Z
  Pref1 : Constant  Value=0.85926
  Pref2 : Constant  Value=1.2473
  Pref3 : Constant  Commented=on  Value=-1.5593
  Pref4 : Constant  Commented=on  Value=9.8766
  Pusat Server Data : spsThreePhaseParallelRLCLoadLib/Three-Phase Parallel RLC Load  LConnTagsString=A|B|C  Configuration=Y (grounded)  NominalVoltage=20e3  Vabc=[1e3 1e3 1e3]  Vabcp=[1e3 1e3 1e3]  NominalFrequency=50  UnbalancedPower=off  ActivePower=2.25e3  InductivePower=1.09e5  CapacitivePower=0  Pabc=[10e3 9e3 11e3]  QLabc=[100 90 110]  QCabc=[100 90 110]  Pabcp=[10e3 9e3 11e3]  QLabcp=[100 90 110]  QCabcp=[100 90 110]  Measurements=Branch voltages and currents  LoadType=constant Z
  RS : spsThreePhaseParallelRLCLoadLib/Three-Phase Parallel RLC Load  LConnTagsString=A|B|C  Configuration=Y (grounded)  NominalVoltage=20e3  Vabc=[1e3 1e3 1e3]  Vabcp=[1e3 1e3 1e3]  NominalFrequency=50  UnbalancedPower=off  ActivePower=9e4  InductivePower=4.36e4  CapacitivePower=0  Pabc=[10e3 9e3 11e3]  QLabc=[100 90 110]  QCabc=[100 90 110]  Pabcp=[10e3 9e3 11e3]  QLabcp=[100 90 110]  QCabcp=[100 90 110]  Measurements=Branch voltages and currents  LoadType=constant Z
  RT1 : spsThreePhaseParallelRLCLoadLib/Three-Phase Parallel RLC Load  Commented=on  LConnTagsString=A|B|C  Configuration=Y (grounded)  NominalVoltage=380  Vabc=[1e3 1e3 1e3]  Vabcp=[1e3 1e3 1e3]  NominalFrequency=50  UnbalancedPower=off  ActivePower=0.88e6  InductivePower=0.389879952e6  CapacitivePower=0  Pabc=[10e3 9e3 11e3]  QLabc=[100 90 110]  QCabc=[100 90 110]  Pabcp=[10e3 9e3 11e3]  QLabcp=[100 90 110]  QCabcp=[100 90 110]  Measurements=Branch voltages and currents  LoadType=constant Z
  RT1.2 : spsThreePhaseParallelRLCLoadLib/Three-Phase Parallel RLC Load  LConnTagsString=A|B|C  Configuration=Y (grounded)  NominalVoltage=380  Vabc=[1e3 1e3 1e3]  Vabcp=[1e3 1e3 1e3]  NominalFrequency=50  UnbalancedPower=off  ActivePower=1.4e6  InductivePower=6.78e5  CapacitivePower=0  Pabc=[10e3 9e3 11e3]  QLabc=[100 90 110]  QCabc=[100 90 110]  Pabcp=[10e3 9e3 11e3]  QLabcp=[100 90 110]  QCabcp=[100 90 110]  Measurements=Branch voltages and currents  LoadType=constant Z
  RT1.3 : spsThreePhaseParallelRLCLoadLib/Three-Phase Parallel RLC Load  Commented=on  LConnTagsString=A|B|C  Configuration=Y (grounded)  NominalVoltage=380  Vabc=[1e3 1e3 1e3]  Vabcp=[1e3 1e3 1e3]  NominalFrequency=50  UnbalancedPower=off  ActivePower=840000  InductivePower=727461.3392  CapacitivePower=0  Pabc=[10e3 9e3 11e3]  QLabc=[100 90 110]  QCabc=[100 90 110]  Pabcp=[10e3 9e3 11e3]  QLabcp=[100 90 110]  QCabcp=[100 90 110]  Measurements=Branch voltages and currents  LoadType=constant Z
  RT2 : spsThreePhaseParallelRLCLoadLib/Three-Phase Parallel RLC Load  Commented=on  LConnTagsString=A|B|C  Configuration=Y (grounded)  NominalVoltage=380  Vabc=[1e3 1e3 1e3]  Vabcp=[1e3 1e3 1e3]  NominalFrequency=50  UnbalancedPower=off  ActivePower=2.8e7  InductivePower=1.36e7  CapacitivePower=0  Pabc=[10e3 9e3 11e3]  QLabc=[100 90 110]  QCabc=[100 90 110]  Pabcp=[10e3 9e3 11e3]  QLabcp=[100 90 110]  QCabcp=[100 90 110]  Measurements=Branch voltages and currents  LoadType=constant Z
  RT2.2 : spsThreePhaseParallelRLCLoadLib/Three-Phase Parallel RLC Load  LConnTagsString=A|B|C  Configuration=Y (grounded)  NominalVoltage=380  Vabc=[1e3 1e3 1e3]  Vabcp=[1e3 1e3 1e3]  NominalFrequency=50  UnbalancedPower=off  ActivePower=2.8e6  InductivePower=1.36e6  CapacitivePower=0  Pabc=[10e3 9e3 11e3]  QLabc=[100 90 110]  QCabc=[100 90 110]  Pabcp=[10e3 9e3 11e3]  QLabcp=[100 90 110]  QCabcp=[100 90 110]  Measurements=Branch voltages and currents  LoadType=constant Z
  RT2.3 : spsThreePhaseParallelRLCLoadLib/Three-Phase Parallel RLC Load  Commented=on  LConnTagsString=A|B|C  Configuration=Y (grounded)  NominalVoltage=380  Vabc=[1e3 1e3 1e3]  Vabcp=[1e3 1e3 1e3]  NominalFrequency=50  UnbalancedPower=off  ActivePower=6000000  InductivePower=4984871.131  CapacitivePower=0  Pabc=[10e3 9e3 11e3]  QLabc=[100 90 110]  QCabc=[100 90 110]  Pabcp=[10e3 9e3 11e3]  QLabcp=[100 90 110]  QCabcp=[100 90 110]  Measurements=Branch voltages and currents  LoadType=constant Z
  RT3 : spsThreePhaseParallelRLCLoadLib/Three-Phase Parallel RLC Load  Commented=on  LConnTagsString=A|B|C  Configuration=Y (grounded)  NominalVoltage=380  Vabc=[1e3 1e3 1e3]  Vabcp=[1e3 1e3 1e3]  NominalFrequency=50  UnbalancedPower=off  ActivePower=1.19e7  InductivePower=5.76e6  CapacitivePower=0  Pabc=[10e3 9e3 11e3]  QLabc=[100 90 110]  QCabc=[100 90 110]  Pabcp=[10e3 9e3 11e3]  QLabcp=[100 90 110]  QCabcp=[100 90 110]  Measurements=Branch voltages and currents  LoadType=constant Z
  RT3.2 : spsThreePhaseParallelRLCLoadLib/Three-Phase Parallel RLC Load  LConnTagsString=A|B|C  Configuration=Y (grounded)  NominalVoltage=380  Vabc=[1e3 1e3 1e3]  Vabcp=[1e3 1e3 1e3]  NominalFrequency=50  UnbalancedPower=off  ActivePower=1.19e6  InductivePower=5.76e6  CapacitivePower=0  Pabc=[10e3 9e3 11e3]  QLabc=[100 90 110]  QCabc=[100 90 110]  Pabcp=[10e3 9e3 11e3]  QLabcp=[100 90 110]  QCabcp=[100 90 110]  Measurements=Branch voltages and currents  LoadType=constant Z
  RT3.3 : spsThreePhaseParallelRLCLoadLib/Three-Phase Parallel RLC Load  Commented=on  LConnTagsString=A|B|C  Configuration=Y (grounded)  NominalVoltage=380  Vabc=[1e3 1e3 1e3]  Vabcp=[1e3 1e3 1e3]  NominalFrequency=50  UnbalancedPower=off  ActivePower=7700000  InductivePower=6483524.479  CapacitivePower=0  Pabc=[10e3 9e3 11e3]  QLabc=[100 90 110]  QCabc=[100 90 110]  Pabcp=[10e3 9e3 11e3]  QLabcp=[100 90 110]  QCabcp=[100 90 110]  Measurements=Branch voltages and currents  LoadType=constant Z
  RT4 : spsThreePhaseParallelRLCLoadLib/Three-Phase Parallel RLC Load  Commented=on  LConnTagsString=A|B|C  Configuration=Y (grounded)  NominalVoltage=380  Vabc=[1e3 1e3 1e3]  Vabcp=[1e3 1e3 1e3]  NominalFrequency=50  UnbalancedPower=off  ActivePower=4.90e6  InductivePower=2.37e6  CapacitivePower=0  Pabc=[10e3 9e3 11e3]  QLabc=[100 90 110]  QCabc=[100 90 110]  Pabcp=[10e3 9e3 11e3]  QLabcp=[100 90 110]  QCabcp=[100 90 110]  Measurements=Branch voltages and currents  LoadType=constant Z
  RT4.2 : spsThreePhaseParallelRLCLoadLib/Three-Phase Parallel RLC Load  LConnTagsString=A|B|C  Configuration=Y (grounded)  NominalVoltage=380  Vabc=[1e3 1e3 1e3]  Vabcp=[1e3 1e3 1e3]  NominalFrequency=50  UnbalancedPower=off  ActivePower=4.9e5  InductivePower=2.37e5  CapacitivePower=0  Pabc=[10e3 9e3 11e3]  QLabc=[100 90 110]  QCabc=[100 90 110]  Pabcp=[10e3 9e3 11e3]  QLabcp=[100 90 110]  QCabcp=[100 90 110]  Measurements=Branch voltages and currents  LoadType=constant Z
  RT4.3 : spsThreePhaseParallelRLCLoadLib/Three-Phase Parallel RLC Load  Commented=on  LConnTagsString=A|B|C  Configuration=Y (grounded)  NominalVoltage=380  Vabc=[1e3 1e3 1e3]  Vabcp=[1e3 1e3 1e3]  NominalFrequency=50  UnbalancedPower=off  ActivePower=3780000  InductivePower=2733433.26  CapacitivePower=0  Pabc=[10e3 9e3 11e3]  QLabc=[100 90 110]  QCabc=[100 90 110]  Pabcp=[10e3 9e3 11e3]  QLabcp=[100 90 110]  QCabcp=[100 90 110]  Measurements=Branch voltages and currents  LoadType=constant Z
  RT5 : spsThreePhaseParallelRLCLoadLib/Three-Phase Parallel RLC Load  Commented=on  LConnTagsString=A|B|C  Configuration=Y (grounded)  NominalVoltage=380  Vabc=[1e3 1e3 1e3]  Vabcp=[1e3 1e3 1e3]  NominalFrequency=50  UnbalancedPower=off  ActivePower=4.20e6  InductivePower=2.03e6  CapacitivePower=0  Pabc=[10e3 9e3 11e3]  QLabc=[100 90 110]  QCabc=[100 90 110]  Pabcp=[10e3 9e3 11e3]  QLabcp=[100 90 110]  QCabcp=[100 90 110]  Measurements=Branch voltages and currents  LoadType=constant Z
  RT5.2 : spsThreePhaseParallelRLCLoadLib/Three-Phase Parallel RLC Load  LConnTagsString=A|B|C  Configuration=Y (grounded)  NominalVoltage=380  Vabc=[1e3 1e3 1e3]  Vabcp=[1e3 1e3 1e3]  NominalFrequency=50  UnbalancedPower=off  ActivePower=4.2e5  InductivePower=2.03e5  CapacitivePower=0  Pabc=[10e3 9e3 11e3]  QLabc=[100 90 110]  QCabc=[100 90 110]  Pabcp=[10e3 9e3 11e3]  QLabcp=[100 90 110]  QCabcp=[100 90 110]  Measurements=Branch voltages and currents  LoadType=constant Z
  RT5.3 : spsThreePhaseParallelRLCLoadLib/Three-Phase Parallel RLC Load  Commented=on  LConnTagsString=A|B|C  Configuration=Y (grounded)  NominalVoltage=380  Vabc=[1e3 1e3 1e3]  Vabcp=[1e3 1e3 1e3]  NominalFrequency=50  UnbalancedPower=off  ActivePower=5280000  InductivePower=3396908.15  CapacitivePower=0  Pabc=[10e3 9e3 11e3]  QLabc=[100 90 110]  QCabc=[100 90 110]  Pabcp=[10e3 9e3 11e3]  QLabcp=[100 90 110]  QCabcp=[100 90 110]  Measurements=Branch voltages and currents  LoadType=constant Z
  Resto-Toko : spsThreePhaseParallelRLCLoadLib/Three-Phase Parallel RLC Load  LConnTagsString=A|B|C  Configuration=Y (grounded)  NominalVoltage=20e3  Vabc=[1e3 1e3 1e3]  Vabcp=[1e3 1e3 1e3]  NominalFrequency=50  UnbalancedPower=off  ActivePower=4.5e5  InductivePower=2.18e5  CapacitivePower=0  Pabc=[10e3 9e3 11e3]  QLabc=[100 90 110]  QCabc=[100 90 110]  Pabcp=[10e3 9e3 11e3]  QLabcp=[100 90 110]  QCabcp=[100 90 110]  Measurements=Branch voltages and currents  LoadType=constant Z
  Rumah Ibadah 2 : spsThreePhaseParallelRLCLoadLib/Three-Phase Parallel RLC Load  LConnTagsString=A|B|C  Configuration=Y (grounded)  NominalVoltage=380  Vabc=[1e3 1e3 1e3]  Vabcp=[1e3 1e3 1e3]  NominalFrequency=50  UnbalancedPower=off  ActivePower=1.19e5  InductivePower=5.75e4  CapacitivePower=0  Pabc=[10e3 9e3 11e3]  QLabc=[100 90 110]  QCabc=[100 90 110]  Pabcp=[10e3 9e3 11e3]  QLabcp=[100 90 110]  QCabcp=[100 90 110]  Measurements=Branch voltages and currents  LoadType=constant Z
  Rumah Ibadah 3 : spsThreePhaseParallelRLCLoadLib/Three-Phase Parallel RLC Load  Commented=on  LConnTagsString=A|B|C  Configuration=Y (grounded)  NominalVoltage=380  Vabc=[1e3 1e3 1e3]  Vabcp=[1e3 1e3 1e3]  NominalFrequency=50  UnbalancedPower=off  ActivePower=0.38016e6  InductivePower=0.11088e6  CapacitivePower=0  Pabc=[10e3 9e3 11e3]  QLabc=[100 90 110]  QCabc=[100 90 110]  Pabcp=[10e3 9e3 11e3]  QLabcp=[100 90 110]  QCabcp=[100 90 110]  Measurements=Branch voltages and currents  LoadType=constant Z
  Rumah ibadah : spsThreePhaseParallelRLCLoadLib/Three-Phase Parallel RLC Load  Commented=on  LConnTagsString=A|B|C  Configuration=Y (grounded)  NominalVoltage=380  Vabc=[1e3 1e3 1e3]  Vabcp=[1e3 1e3 1e3]  NominalFrequency=50  UnbalancedPower=off  ActivePower=1.188e6  InductivePower=0.5753746605e6  CapacitivePower=0  Pabc=[10e3 9e3 11e3]  QLabc=[100 90 110]  QCabc=[100 90 110]  Pabcp=[10e3 9e3 11e3]  QLabcp=[100 90 110]  QCabcp=[100 90 110]  Measurements=Branch voltages and currents  LoadType=constant Z
  Scope : Scope
  Three-Phase Breaker{,1..4,8,11..13,24..28,30,32..34} (18 alike) : spsThreePhaseBreakerLib/Three-Phase Breaker  Commented=on  InitialState=closed  SwitchA=off  SwitchB=off  SwitchC=off  SwitchTimes="[4/10  13/10]"  External=off  BreakerResistance=0.01  SnubberResistance=1e6  SnubberCapacitance=inf  Measurements=None
  Three-Phase Breaker{5..7,9..10,14..23,29,31} (17 alike) : spsThreePhaseBreakerLib/Three-Phase Breaker  InitialState=closed  SwitchA=off  SwitchB=off  SwitchC=off  SwitchTimes="[4/10  13/10]"  External=off  BreakerResistance=0.01  SnubberResistance=1e6  SnubberCapacitance=inf  Measurements=None
  Trafo 1 SD 20:0.38 : spsThreePhaseTransformerTwoWindingsLib/Three-Phase Transformer (Two Windings)  Winding1Connection=Yg  Winding2Connection=Yg  CoreType=Three single-phase transformers  SetSaturation=off  Hysteresis=off  DataFile='hysteresis'  SetInitialFlux=off  Measurements=None  UNITS=pu  NominalPower=[ 250e6 , 50 ]  Winding1=[20000 0.005 0]  Winding2=[380 0.005 3.18e-4]  Rm=500  Lm=500  L0=0.5  Saturation=[0 0;0.0024001 1.2;0.99999 1.52]  InitialFluxes=[0.8 -0.8 0.7]  BreakLoop=off  DiscreteSolver=Trapezoidal iterative  DataType=off  TransfoNumber=1
  Trafo 1 SD 70:20 : spsThreePhaseTransformerTwoWindingsLib/Three-Phase Transformer (Two Windings)  Winding1Connection=Delta (D1)  Winding2Connection=Yg  CoreType=Three single-phase transformers  SetSaturation=off  Hysteresis=off  DataFile='hysteresis'  SetInitialFlux=off  Measurements=None  UNITS=pu  NominalPower=[ 250e6 , 50 ]  Winding1=[ 70e3 , 0.005 , 3.18e-4 ]  Winding2=[ 20e3 , 0.005 , 0 ]  Rm=500  Lm=500  L0=0.5  Saturation=[ 0,0 ; 0.0024,1.2 ; 1.0,1.52 ]  InitialFluxes=[ 0.8 , -0.8 , 0.7 ]  BreakLoop=off  DiscreteSolver=Trapezoidal iterative  DataType=off  TransfoNumber=1
  Trafo 1 SU 20:70 : spsThreePhaseTransformerTwoWindingsLib/Three-Phase Transformer (Two Windings)  Winding1Connection=Yg  Winding2Connection=Delta (D1)  CoreType=Three single-phase transformers  SetSaturation=off  Hysteresis=off  DataFile='hysteresis'  SetInitialFlux=off  Measurements=None  UNITS=pu  NominalPower=[ 250e6 , 50 ]  Winding1=[20000 0.005 0]  Winding2=[70000 0.005 3.18e-4]  Rm=500  Lm=500  L0=0.5  Saturation=[0 0;0.0024001 1.2;0.99999 1.52]  InitialFluxes=[0.8 -0.8 0.7]  BreakLoop=off  DiscreteSolver=Trapezoidal iterative  DataType=off  TransfoNumber=1
  Trafo 1 SU 230:70 : spsThreePhaseTransformerTwoWindingsLib/Three-Phase Transformer (Two Windings)  Winding1Connection=Yg  Winding2Connection=Delta (D1)  CoreType=Three single-phase transformers  SetSaturation=off  Hysteresis=off  DataFile='hysteresis'  SetInitialFlux=off  Measurements=None  UNITS=pu  NominalPower=[ 250e6 , 50 ]  Winding1=[ 230e3 , 0.005 , 3.18e-4 ]  Winding2=[ 70e3 , 0.005 , 0 ]  Rm=500  Lm=500  L0=0.5  Saturation=[ 0,0 ; 0.0024,1.2 ; 1.0,1.52 ]  InitialFluxes=[ 0.8 , -0.8 , 0.7 ]  BreakLoop=off  DiscreteSolver=Trapezoidal iterative  DataType=off  TransfoNumber=1
  Trafo 1 SU 70:230 : spsThreePhaseTransformerTwoWindingsLib/Three-Phase Transformer (Two Windings)  Winding1Connection=Delta (D1)  Winding2Connection=Yg  CoreType=Three single-phase transformers  SetSaturation=off  Hysteresis=off  DataFile='hysteresis'  SetInitialFlux=off  Measurements=None  UNITS=pu  NominalPower=[ 250e6 , 50 ]  Winding1=[70000 0.005 0]  Winding2=[230000 0.005 3.18e-4]  Rm=500  Lm=500  L0=0.5  Saturation=[0 0;0.0024001 1.2;0.99999 1.52]  InitialFluxes=[0.8 -0.8 0.7]  BreakLoop=off  DiscreteSolver=Trapezoidal iterative  DataType=off  TransfoNumber=1
  Trafo 2 SD 70:20 : spsThreePhaseTransformerTwoWindingsLib/Three-Phase Transformer (Two Windings)  Winding1Connection=Delta (D1)  Winding2Connection=Yg  CoreType=Three single-phase transformers  SetSaturation=off  Hysteresis=off  DataFile='hysteresis'  SetInitialFlux=off  Measurements=None  UNITS=pu  NominalPower=[ 250e6 , 50 ]  Winding1=[ 70e3 , 0.005 , 3.18e-4 ]  Winding2=[ 20e3 , 0.005 , 0 ]  Rm=500  Lm=500  L0=0.5  Saturation=[ 0,0 ; 0.0024,1.2 ; 1.0,1.52 ]  InitialFluxes=[ 0.8 , -0.8 , 0.7 ]  BreakLoop=off  DiscreteSolver=Trapezoidal iterative  DataType=off  TransfoNumber=1
  Trafo 2 SU 20:70 : spsThreePhaseTransformerTwoWindingsLib/Three-Phase Transformer (Two Windings)  Winding1Connection=Yg  Winding2Connection=Delta (D1)  CoreType=Three single-phase transformers  SetSaturation=off  Hysteresis=off  DataFile='hysteresis'  SetInitialFlux=off  Measurements=None  UNITS=pu  NominalPower=[ 250e6 , 50 ]  Winding1=[20000 0.005 0]  Winding2=[70000 0.005 3.18e-4]  Rm=500  Lm=500  L0=0.5  Saturation=[0 0;0.0024001 1.2;0.99999 1.52]  InitialFluxes=[0.8 -0.8 0.7]  BreakLoop=off  DiscreteSolver=Trapezoidal iterative  DataType=off  TransfoNumber=1
  Trafo 2 SU 230:70 : spsThreePhaseTransformerTwoWindingsLib/Three-Phase Transformer (Two Windings)  Winding1Connection=Yg  Winding2Connection=Delta (D1)  CoreType=Three single-phase transformers  SetSaturation=off  Hysteresis=off  DataFile='hysteresis'  SetInitialFlux=off  Measurements=None  UNITS=pu  NominalPower=[ 250e6 , 50 ]  Winding1=[ 230e3 , 0.005 , 3.18e-4 ]  Winding2=[ 70e3 , 0.005 , 0 ]  Rm=500  Lm=500  L0=0.5  Saturation=[ 0,0 ; 0.0024,1.2 ; 1.0,1.52 ]  InitialFluxes=[ 0.8 , -0.8 , 0.7 ]  BreakLoop=off  DiscreteSolver=Trapezoidal iterative  DataType=off  TransfoNumber=1
  Trafo 2 SU 70:230 : spsThreePhaseTransformerTwoWindingsLib/Three-Phase Transformer (Two Windings)  Winding1Connection=Delta (D1)  Winding2Connection=Yg  CoreType=Three single-phase transformers  SetSaturation=off  Hysteresis=off  DataFile='hysteresis'  SetInitialFlux=off  Measurements=None  UNITS=pu  NominalPower=[ 250e6 , 50 ]  Winding1=[70000 0.005 0]  Winding2=[230000 0.005 3.18e-4]  Rm=500  Lm=500  L0=0.5  Saturation=[0 0;0.0024001 1.2;0.99999 1.52]  InitialFluxes=[0.8 -0.8 0.7]  BreakLoop=off  DiscreteSolver=Trapezoidal iterative  DataType=off  TransfoNumber=1
  Trafo 3 SD 70:20 : spsThreePhaseTransformerTwoWindingsLib/Three-Phase Transformer (Two Windings)  Winding1Connection=Delta (D1)  Winding2Connection=Yg  CoreType=Three single-phase transformers  SetSaturation=off  Hysteresis=off  DataFile='hysteresis'  SetInitialFlux=off  Measurements=None  UNITS=pu  NominalPower=[ 250e6 , 50 ]  Winding1=[ 70e3 , 0.005 , 3.18e-4 ]  Winding2=[ 20e3 , 0.005 , 0 ]  Rm=500  Lm=500  L0=0.5  Saturation=[ 0,0 ; 0.0024,1.2 ; 1.0,1.52 ]  InitialFluxes=[ 0.8 , -0.8 , 0.7 ]  BreakLoop=off  DiscreteSolver=Trapezoidal iterative  DataType=off  TransfoNumber=1
  Trafo 3 SU 20:70 : spsThreePhaseTransformerTwoWindingsLib/Three-Phase Transformer (Two Windings)  Commented=on  Winding1Connection=Yg  Winding2Connection=Delta (D1)  CoreType=Three single-phase transformers  SetSaturation=off  Hysteresis=off  DataFile='hysteresis'  SetInitialFlux=off  Measurements=None  UNITS=pu  NominalPower=[ 250e6 , 50 ]  Winding1=[20000 0.005 0]  Winding2=[70000 0.005 3.18e-4]  Rm=500  Lm=500  L0=0.5  Saturation=[0 0;0.0024001 1.2;0.99999 1.52]  InitialFluxes=[0.8 -0.8 0.7]  BreakLoop=off  DiscreteSolver=Trapezoidal iterative  DataType=off  TransfoNumber=1
  Trafo 3 SU 230:70 : spsThreePhaseTransformerTwoWindingsLib/Three-Phase Transformer (Two Windings)  Commented=on  Winding1Connection=Yg  Winding2Connection=Delta (D1)  CoreType=Three single-phase transformers  SetSaturation=off  Hysteresis=off  DataFile='hysteresis'  SetInitialFlux=off  Measurements=None  UNITS=pu  NominalPower=[ 250e6 , 50 ]  Winding1=[ 230e3 , 0.005 , 3.18e-4 ]  Winding2=[ 70e3 , 0.005 , 0 ]  Rm=500  Lm=500  L0=0.5  Saturation=[ 0,0 ; 0.0024,1.2 ; 1.0,1.52 ]  InitialFluxes=[ 0.8 , -0.8 , 0.7 ]  BreakLoop=off  DiscreteSolver=Trapezoidal iterative  DataType=off  TransfoNumber=1
  Trafo 3 SU 70:230 : spsThreePhaseTransformerTwoWindingsLib/Three-Phase Transformer (Two Windings)  Commented=on  Winding1Connection=Delta (D1)  Winding2Connection=Yg  CoreType=Three single-phase transformers  SetSaturation=off  Hysteresis=off  DataFile='hysteresis'  SetInitialFlux=off  Measurements=None  UNITS=pu  NominalPower=[ 250e6 , 50 ]  Winding1=[70000 0.005 0]  Winding2=[230000 0.005 3.18e-4]  Rm=500  Lm=500  L0=0.5  Saturation=[0 0;0.0024001 1.2;0.99999 1.52]  InitialFluxes=[0.8 -0.8 0.7]  BreakLoop=off  DiscreteSolver=Trapezoidal iterative  DataType=off  TransfoNumber=1
  Trafo 4 SD 70:20 : spsThreePhaseTransformerTwoWindingsLib/Three-Phase Transformer (Two Windings)  Winding1Connection=Delta (D1)  Winding2Connection=Yg  CoreType=Three single-phase transformers  SetSaturation=off  Hysteresis=off  DataFile='hysteresis'  SetInitialFlux=off  Measurements=None  UNITS=pu  NominalPower=[ 250e6 , 50 ]  Winding1=[ 70e3 , 0.005 , 3.18e-4 ]  Winding2=[ 20e3 , 0.005 , 0 ]  Rm=500  Lm=500  L0=0.5  Saturation=[ 0,0 ; 0.0024,1.2 ; 1.0,1.52 ]  InitialFluxes=[ 0.8 , -0.8 , 0.7 ]  BreakLoop=off  DiscreteSolver=Trapezoidal iterative  DataType=off  TransfoNumber=1
  Trafo 4 SU 20:70 : spsThreePhaseTransformerTwoWindingsLib/Three-Phase Transformer (Two Windings)  Commented=on  Winding1Connection=Yg  Winding2Connection=Delta (D1)  CoreType=Three single-phase transformers  SetSaturation=off  Hysteresis=off  DataFile='hysteresis'  SetInitialFlux=off  Measurements=None  UNITS=pu  NominalPower=[ 250e6 , 50 ]  Winding1=[20000 0.005 0]  Winding2=[70000 0.005 3.18e-4]  Rm=500  Lm=500  L0=0.5  Saturation=[0 0;0.0024001 1.2;0.99999 1.52]  InitialFluxes=[0.8 -0.8 0.7]  BreakLoop=off  DiscreteSolver=Trapezoidal iterative  DataType=off  TransfoNumber=1
  Trafo 4 SU 230:70 : spsThreePhaseTransformerTwoWindingsLib/Three-Phase Transformer (Two Windings)  Commented=on  Winding1Connection=Yg  Winding2Connection=Delta (D1)  CoreType=Three single-phase transformers  SetSaturation=off  Hysteresis=off  DataFile='hysteresis'  SetInitialFlux=off  Measurements=None  UNITS=pu  NominalPower=[ 250e6 , 50 ]  Winding1=[ 230e3 , 0.005 , 3.18e-4 ]  Winding2=[ 70e3 , 0.005 , 0 ]  Rm=500  Lm=500  L0=0.5  Saturation=[ 0,0 ; 0.0024,1.2 ; 1.0,1.52 ]  InitialFluxes=[ 0.8 , -0.8 , 0.7 ]  BreakLoop=off  DiscreteSolver=Trapezoidal iterative  DataType=off  TransfoNumber=1
  Trafo 4 SU 70:1 : spsThreePhaseTransformerTwoWindingsLib/Three-Phase Transformer (Two Windings)  Commented=on  Winding1Connection=Delta (D1)  Winding2Connection=Yg  CoreType=Three single-phase transformers  SetSaturation=off  Hysteresis=off  DataFile='hysteresis'  SetInitialFlux=off  Measurements=None  UNITS=pu  NominalPower=[ 250e6 , 50 ]  Winding1=[70000 0.005 0]  Winding2=[230000 0.005 3.18e-4]  Rm=500  Lm=500  L0=0.5  Saturation=[0 0;0.0024001 1.2;0.99999 1.52]  InitialFluxes=[0.8 -0.8 0.7]  BreakLoop=off  DiscreteSolver=Trapezoidal iterative  DataType=off  TransfoNumber=1
  Trafo 5 SD 20:0.38 : spsThreePhaseTransformerTwoWindingsLib/Three-Phase Transformer (Two Windings)  Winding1Connection=Yg  Winding2Connection=Yg  CoreType=Three single-phase transformers  SetSaturation=off  Hysteresis=off  DataFile='hysteresis'  SetInitialFlux=off  Measurements=None  UNITS=pu  NominalPower=[ 250e6 , 50 ]  Winding1=[ 20e3 , 0.005 , 0 ]  Winding2=[ 380, 0.005 , 3.18e-4 ]  Rm=500  Lm=500  L0=0.5  Saturation=[0 0;0.0024 1.2;0.99999 1.52]  InitialFluxes=[0.8 -0.8 0.7]  BreakLoop=off  DiscreteSolver=Trapezoidal iterative  DataType=off  TransfoNumber=1
  UKM : spsThreePhaseParallelRLCLoadLib/Three-Phase Parallel RLC Load  Commented=on  LConnTagsString=A|B|C  Configuration=Y (grounded)  NominalVoltage=20e3  Vabc=[1e3 1e3 1e3]  Vabcp=[1e3 1e3 1e3]  NominalFrequency=50  UnbalancedPower=off  ActivePower=5.85e6  InductivePower=2.83e6  CapacitivePower=0  Pabc=[10e3 9e3 11e3]  QLabc=[100 90 110]  QCabc=[100 90 110]  Pabcp=[10e3 9e3 11e3]  QLabcp=[100 90 110]  QCabcp=[100 90 110]  Measurements=Branch voltages and currents  LoadType=constant Z
  Univ - Sekolah : spsThreePhaseParallelRLCLoadLib/Three-Phase Parallel RLC Load  Commented=on  LConnTagsString=A|B|C  Configuration=Y (grounded)  NominalVoltage=380  Vabc=[1e3 1e3 1e3]  Vabcp=[1e3 1e3 1e3]  NominalFrequency=50  UnbalancedPower=off  ActivePower=0.9e6  InductivePower=0.4358898944e6  CapacitivePower=0  Pabc=[10e3 9e3 11e3]  QLabc=[100 90 110]  QCabc=[100 90 110]  Pabcp=[10e3 9e3 11e3]  QLabcp=[100 90 110]  QCabcp=[100 90 110]  Measurements=Branch voltages and currents  LoadType=constant Z
  Univ - Sekolah 2 : spsThreePhaseParallelRLCLoadLib/Three-Phase Parallel RLC Load  Commented=on  LConnTagsString=A|B|C  Configuration=Y (grounded)  NominalVoltage=380  Vabc=[1e3 1e3 1e3]  Vabcp=[1e3 1e3 1e3]  NominalFrequency=50  UnbalancedPower=off  ActivePower=0.54e6  InductivePower=0.2615339366e6  CapacitivePower=0  Pabc=[10e3 9e3 11e3]  QLabc=[100 90 110]  QCabc=[100 90 110]  Pabcp=[10e3 9e3 11e3]  QLabcp=[100 90 110]  QCabcp=[100 90 110]  Measurements=Branch voltages and currents  LoadType=constant Z
  Univ - Sekolah 3 : spsThreePhaseParallelRLCLoadLib/Three-Phase Parallel RLC Load  Commented=on  LConnTagsString=A|B|C  Configuration=Y (grounded)  NominalVoltage=380  Vabc=[1e3 1e3 1e3]  Vabcp=[1e3 1e3 1e3]  NominalFrequency=50  UnbalancedPower=off  ActivePower=0.288e6  InductivePower=0.084e6  CapacitivePower=0  Pabc=[10e3 9e3 11e3]  QLabc=[100 90 110]  QCabc=[100 90 110]  Pabcp=[10e3 9e3 11e3]  QLabcp=[100 90 110]  QCabcp=[100 90 110]  Measurements=Branch voltages and currents  LoadType=constant Z
  Vref1 : Constant
  Vref2 : Constant
  Vref3 : Constant  Commented=on
  Vref4 : Constant  Commented=on
  "powergui " : spspowerguiLib/powergui  Priority=1  SimulationMode=Continuous  SampleTime=50e-6  frequency=50  Iterations=100  frequencyindice=50  Pbase=100e6  ErrMax=1e-4  UnitsV=kV  UnitsW=MW  buscounter=0  FunctionMessages=off  echomessages=off  EnableUseOfTLC=off  CurrentSourceSwitches=off  DisableSnubberDevices=off  DisableRonSwitches=off  DisableVfSwitches=off  DisplayEquations=off  AutomaticDiscreteSolvers=off  SolverType=Tustin  Interpol=off  ExternalGateDelay=off  methode=off  Ts=0  x0status=blocks  SPID=off  SwTol=0  HookPort=off  NonlinearTolerance=1e-4  nMaxIteration=100  ContinueOnMaxIteration=off  RestoreLinks=warning  ResistiveCurrentMeasurement=off  Frange=[0:2:500]  Ylog=off  Xlog=on  ShowGrid=off  save=off  variable=ZData  structure=0  ZoomFFT=off  StartTime=0.0  cycles=1  DisplayStyle=1  fundamental=60  FreqAxis=off  MaxFrequency=1000  frequencyindicesteady=1  RmsSteady=1  display=off
  wires:
  Multimeter/1 -> Scope/1
  PLTP/1 -> Bus Selector/1
  Vref1/1 -> Excitation System 1/1
  Excitation System 1/1 -> PLTP/2
  Bus Selector/1 -> Excitation System 1/3  "<Stator voltage  vq (pu)>"
  Bus Selector/2 -> Excitation System 1/2  "<Stator voltage  vd (pu)>"
  Pref1/1 -> PLTP/1
  Bus Selector1/2 -> Excitation System 2/2  "<Stator voltage  vd (pu)>"
  Bus Selector1/1 -> Excitation System 2/3  "<Stator voltage  vq (pu)>"
  PLTU/1 -> Bus Selector1/1
  Pref2/1 -> PLTU/1
  Vref2/1 -> Excitation System 2/1
  Excitation System 2/1 -> PLTU/2
  Bus Selector2/1 -> Excitation System 3/3  "<Stator voltage  vq (pu)>"
  Pref3/1 -> PLTA/1
  Vref3/1 -> Excitation System 3/1
  Excitation System 3/1 -> PLTA/2
  Bus Selector2/2 -> Excitation System 3/2  "<Stator voltage  vd (pu)>"
  PLTA/1 -> Bus Selector2/1
  Pref4/1 -> PLTB/1
  Vref4/1 -> Excitation System 4/1
  Excitation System 4/1 -> PLTB/2
  Bus Selector3/1 -> Excitation System 4/3  "<Stator voltage  vq (pu)>"
  PLTB/1 -> Bus Selector3/1
  Bus Selector3/2 -> Excitation System 4/2  "<Stator voltage  vd (pu)>"
  connections:
  CB 21-22/LConn3 -- Trafo 2 SU 20:70/RConn3
  CB 11-12/RConn2 -- Trafo 1 SU 70:230/LConn2 -- CB 11-1/RConn2
  CB 24-Gardu 2/LConn2 -- Trafo 2 SU 230:70/RConn2
  CB 11-12/LConn2 -- Trafo 1 SU 20:70/RConn2
  CB L2-4/LConn3 -- Line 2-4/LConn3
  CB 45-46/LConn1 -- Trafo 4 SD 70:20/RConn1
  CB L1-3/RConn3 -- Trafo 1 SD 70:20/LConn3 -- CB L1-2/RConn3 -- CB 14-Gardu 1/RConn3 -- CB L1-4/RConn3
  CB 11-12/RConn1 -- Trafo 1 SU 70:230/LConn1 -- CB 11-1/RConn1
  Line 1-4/RConn3 -- CB L4-1/RConn3
  CB 11-12/LConn1 -- Trafo 1 SU 20:70/RConn1
  Line 2-4/LConn1 -- CB L2-4/LConn1
  CB 45-46/LConn3 -- Trafo 4 SD 70:20/RConn3
  Line 1-1/LConn3 -- CB L1-2/LConn3
  CB 24-Gardu 2/LConn1 -- Trafo 2 SU 230:70/RConn1
  CB 15-16/LConn1 -- Trafo 1 SD 70:20/RConn1
  CB 13-14/RConn3 -- Trafo 1 SU 230:70/LConn3
  Trafo 1 SU 230:70/RConn3 -- CB 14-Gardu 1/LConn3
  CB L1-3/RConn2 -- Trafo 1 SD 70:20/LConn2 -- CB L1-2/RConn2 -- CB 14-Gardu 1/RConn2 -- CB L1-4/RConn2
  CB 14-Gardu 1/LConn1 -- Trafo 1 SU 230:70/RConn1
  Line 1-1/LConn2 -- CB L1-2/LConn2
  Line 1-1/RConn2 -- CB L2-1/RConn2
  Line 2-3/RConn1 -- CB L3-2/RConn1
  CB 21-22/RConn2 -- Trafo 2 SU 70:230/LConn2 -- CB 11-1/LConn2
  Line 1-3/RConn2 -- CB L3-1/RConn2
  CB 13-14/RConn2 -- Trafo 1 SU 230:70/LConn2
  CB 21-22/LConn1 -- Trafo 2 SU 20:70/RConn1
  CB L4-2/LConn2 -- CB L4-1/LConn2 -- Trafo 4 SD 70:20/LConn2 -- CB L4-3/LConn2 -- CB 44-Gardu 4/RConn2
  CB L1-3/LConn3 -- Line 1-3/LConn3
  CB 14-Gardu 1/LConn2 -- Trafo 1 SU 230:70/RConn2
  CB 11-12/RConn3 -- CB 11-1/RConn3 -- Trafo 1 SU 70:230/LConn3
  Line 3-4/LConn2 -- CB L3-4/LConn2
  Line 2-3/RConn3 -- CB L3-2/RConn3
  Line 3-4/LConn1 -- CB L3-4/LConn1
  Trafo 2 SU 20:70/LConn3 -- CB PLTU-1/RConn3
  Line 3-4/RConn2 -- CB L4-3/RConn2
  Line 2-4/RConn2 -- CB L4-2/RConn2
  CB 15-16/LConn2 -- Trafo 1 SD 70:20/RConn2
  Line 1-3/LConn2 -- CB L1-3/LConn2
  CB L1-3/RConn1 -- Trafo 1 SD 70:20/LConn1 -- CB L1-2/RConn1 -- CB 14-Gardu 1/RConn1 -- CB L1-4/RConn1
  Line 1-3/RConn3 -- CB L3-1/RConn3
  Line 2-4/LConn2 -- CB L2-4/LConn2
  Line 1-3/RConn1 -- CB L3-1/RConn1
  CB L1-4/LConn3 -- Line 1-4/LConn3
  Line 1-1/RConn3 -- CB L2-1/RConn3
  Line 2-4/RConn3 -- CB L4-2/RConn3
  Line 2-3/RConn2 -- CB L3-2/RConn2
  CB PLTU-1/RConn1 -- Trafo 2 SU 20:70/LConn1
  CB L4-1/LConn1 -- CB L4-2/LConn1 -- CB 44-Gardu 4/RConn1 -- CB L4-3/LConn1 -- Trafo 4 SD 70:20/LConn1
  Line 1-1/LConn1 -- CB L1-2/LConn1
  CB PLTP-1/RConn3 -- Trafo 1 SU 20:70/LConn3
  CB L4-1/LConn3 -- CB 44-Gardu 4/RConn3 -- CB L4-2/LConn3 -- Trafo 4 SD 70:20/LConn3 -- CB L4-3/LConn3
  CB 21-22/LConn2 -- Trafo 2 SU 20:70/RConn2
  Trafo 2 SU 230:70/RConn3 -- CB 24-Gardu 2/LConn3
  Line 2-3/LConn2 -- CB L2-3/LConn2
  Line 1-4/LConn1 -- CB L1-4/LConn1
  CB PLTU-1/RConn2 -- Trafo 2 SU 20:70/LConn2
  CB 13-14/RConn1 -- Trafo 1 SU 230:70/LConn1
  Line 1-4/RConn2 -- CB L4-1/RConn2
  Cap Bank RT1/LConn1 -- CB 16-15/LConn1 -- CB 15-16/RConn1
  CB 21-22/RConn1 -- CB 11-1/LConn1 -- Trafo 2 SU 70:230/LConn1
  CB L3-4/LConn3 -- Line 3-4/LConn3
  CB PLTP-1/RConn1 -- Trafo 1 SU 20:70/LConn1
  Line 2-3/LConn1 -- CB L2-3/LConn1
  CB PLTP-1/RConn2 -- Trafo 1 SU 20:70/LConn2
  Line 3-4/RConn1 -- CB L4-3/RConn1
  CB 23-22/LConn2 -- Trafo 2 SU 70:230/RConn2
  CB 11-12/LConn3 -- Trafo 1 SU 20:70/RConn3
  Line 1-3/LConn1 -- CB L1-3/LConn1
  Line 1-4/RConn1 -- CB L4-1/RConn1
  CB 45-46/LConn2 -- Trafo 4 SD 70:20/RConn2
  Line 1-1/RConn1 -- CB L2-1/RConn1
  CB 23-24/RConn2 -- Trafo 2 SU 230:70/LConn2
  CB L2-3/LConn3 -- Line 2-3/LConn3
  Trafo 1 SD 70:20/RConn3 -- CB 15-16/LConn3
  Line 3-4/RConn3 -- CB L4-3/RConn3
  Line 2-4/RConn1 -- CB L4-2/RConn1
  CB 21-22/RConn3 -- Trafo 2 SU 70:230/LConn3 -- CB 11-1/LConn3
  Line 1-4/LConn2 -- CB L1-4/LConn2
  Cap Bank RT1/LConn3 -- CB 16-15/LConn3 -- CB 15-16/RConn3
  CB PLTA-1/RConn2 -- Trafo 3 SU 20:70/LConn2
  CB 31-32/LConn1 -- Trafo 3 SU 20:70/RConn1
  CB 31-32/RConn1 -- Trafo 3 SU 70:230/LConn1
  CB 34-Gardu 3/LConn2 -- Trafo 3 SU 230:70/RConn2
  CB 31-32/LConn3 -- Trafo 3 SU 20:70/RConn3
  CB 34-Gardu 3/LConn1 -- Trafo 3 SU 230:70/RConn1
  CB 31-32/RConn2 -- Trafo 3 SU 70:230/LConn2
  CB 31-32/LConn2 -- Trafo 3 SU 20:70/RConn2
  CB PLTA-1/RConn3 -- Trafo 3 SU 20:70/LConn3
  CB 31-32/RConn3 -- Trafo 3 SU 70:230/LConn3
  CB PLTA-1/RConn1 -- Trafo 3 SU 20:70/LConn1
  Trafo 3 SU 230:70/RConn3 -- CB 34-Gardu 3/LConn3
  CB PLTB-1/RConn1 -- Trafo 4 SU 20:70/LConn1
  CB 41-42/LConn2 -- Trafo 4 SU 20:70/RConn2
  CB 41-42/RConn2 -- Trafo 4 SU 70:1/LConn2
  CB PLTB-1/RConn3 -- Trafo 4 SU 20:70/LConn3
  CB 44-Gardu 4/LConn1 -- Trafo 4 SU 230:70/RConn1
  CB 44-Gardu 4/LConn2 -- Trafo 4 SU 230:70/RConn2
  CB 41-42/LConn1 -- Trafo 4 SU 20:70/RConn1
  CB 41-42/RConn1 -- Trafo 4 SU 70:1/LConn1
  CB 43-44/RConn3 -- Trafo 4 SU 230:70/LConn3
  CB 43-44/RConn2 -- Trafo 4 SU 230:70/LConn2
  CB 41-42/LConn3 -- Trafo 4 SU 20:70/RConn3
  CB PLTB-1/RConn2 -- Trafo 4 SU 20:70/LConn2
  Trafo 4 SU 230:70/RConn3 -- CB 44-Gardu 4/LConn3
  CB 41-42/RConn3 -- Trafo 4 SU 70:1/LConn3
  CB 43-44/RConn1 -- Trafo 4 SU 230:70/LConn1
  CB PLTP-1/LConn1 -- PLTP/RConn1
  CB PLTP-1/LConn3 -- PLTP/RConn3
  CB PLTP-1/LConn2 -- PLTP/RConn2
  CB PLTU-1/LConn3 -- PLTU/RConn3
  CB PLTU-1/LConn2 -- PLTU/RConn2
  CB PLTU-1/LConn1 -- PLTU/RConn1
  CB PLTA-1/LConn2 -- PLTA/RConn2
  CB PLTA-1/LConn3 -- PLTA/RConn3
  CB PLTA-1/LConn1 -- PLTA/RConn1
  CB PLTB-1/LConn1 -- PLTB/RConn1
  CB PLTB-1/LConn3 -- PLTB/RConn3
  CB PLTB-1/LConn2 -- PLTB/RConn2
  CB 16-15/LConn2 -- CB 15-16/RConn2 -- Cap Bank RT1/LConn2
  Line beban 1/RConn3 -- Line beban 6/RConn3 -- Line beban 5/RConn3 -- CB 16-17/LConn3 -- Line beban 3/RConn3 -- Line beban 2/RConn3
  CB 16-15/RConn3 -- Line beban 2/LConn3 -- Line beban 1/LConn3 -- Line beban 6/LConn3 -- Line beban 5/LConn3 -- Line beban 3/LConn3
  CB 16-15/RConn1 -- Line beban 2/LConn1 -- Line beban 1/LConn1 -- Line beban 6/LConn1 -- Line beban 5/LConn1 -- Line beban 3/LConn1
  CB 16-15/RConn2 -- Line beban 2/LConn2 -- Line beban 1/LConn2 -- Line beban 6/LConn2 -- Line beban 5/LConn2 -- Line beban 3/LConn2
  Line beban 1/RConn1 -- Line beban 6/RConn1 -- Line beban 5/RConn1 -- CB 16-17/LConn1 -- Line beban 3/RConn1 -- Line beban 2/RConn1
  Line beban 1/RConn2 -- Line beban 6/RConn2 -- Line beban 5/RConn2 -- CB 16-17/LConn2 -- Line beban 3/RConn2 -- Line beban 2/RConn2
  Three-Phase Breaker/RConn3 -- RT1/LConn3
  Trafo 1 SD 20:0.38/RConn3 -- CB 17-beban/LConn3
  Three-Phase Breaker3/RConn1 -- RT4/LConn1
  CB 16-17/RConn3 -- Trafo 1 SD 20:0.38/LConn3
  Three-Phase Breaker2/RConn3 -- RT3/LConn3
  Three-Phase Breaker/RConn1 -- RT1/LConn1
  Three-Phase Breaker2/RConn1 -- RT3/LConn1
  Three-Phase Breaker2/RConn2 -- RT3/LConn2
  Three-Phase Breaker/RConn2 -- RT1/LConn2
  Three-Phase Breaker3/RConn3 -- RT4/LConn3
  Three-Phase Breaker4/RConn1 -- RT5/LConn1
  Three-Phase Breaker4/RConn2 -- RT5/LConn2
  Three-Phase Breaker1/RConn3 -- RT2/LConn3
  Trafo 1 SD 20:0.38/RConn1 -- CB 17-beban/LConn1
  Three-Phase Breaker1/RConn2 -- RT2/LConn2
  CB 16-17/RConn2 -- Trafo 1 SD 20:0.38/LConn2
  CB 16-17/RConn1 -- Trafo 1 SD 20:0.38/LConn1
  Three-Phase Breaker3/RConn2 -- RT4/LConn2
  Three-Phase Breaker1/RConn1 -- RT2/LConn1
  CB 17-beban/LConn2 -- Trafo 1 SD 20:0.38/RConn2
  Three-Phase Breaker4/RConn3 -- RT5/LConn3
  Three-Phase Breaker7/RConn1 -- Industri besar/LConn1
  CB 25-beban/LConn1 -- Trafo 2 SD 70:20/RConn1
  Three-Phase Breaker9/RConn2 -- Resto-Toko/LConn2
  Three-Phase Breaker10/RConn3 -- Mall-Hotel/LConn3
  Three-Phase Breaker9/RConn1 -- Resto-Toko/LConn1
  Three-Phase Breaker8/RConn1 -- UKM/LConn1
  Three-Phase Breaker10/RConn2 -- Mall-Hotel/LConn2
  Three-Phase Breaker7/RConn3 -- Industri besar/LConn3
  Three-Phase Breaker8/RConn2 -- UKM/LConn2
  Three-Phase Breaker9/RConn3 -- Resto-Toko/LConn3
  Three-Phase Breaker6/RConn3 -- Industri sedang/LConn3
  Three-Phase Breaker5/RConn2 -- Industri kecil/LConn2
  Three-Phase Breaker5/RConn1 -- Industri kecil/LConn1
  Three-Phase Breaker8/RConn3 -- UKM/LConn3
  Three-Phase Breaker7/RConn2 -- Industri besar/LConn2
  CB L2-4/RConn1 -- Trafo 2 SD 70:20/LConn1 -- CB L2-3/RConn1 -- CB L2-1/LConn1 -- CB 24-Gardu 2/RConn1
  Three-Phase Breaker5/LConn2 -- Three-Phase Breaker8/LConn2 -- Three-Phase Breaker9/LConn2 -- Three-Phase Breaker10/LConn2 -- Three-Phase Breaker7/LConn2 -- Cap Bank RT2/LConn2 -- CB 25-beban/RConn2 -- Three-Phase Breaker6/LConn2
  Three-Phase Breaker6/RConn1 -- Industri sedang/LConn1
  Three-Phase Breaker10/RConn1 -- Mall-Hotel/LConn1
  CB L2-3/RConn2 -- Trafo 2 SD 70:20/LConn2 -- CB L2-1/LConn2 -- CB 24-Gardu 2/RConn2 -- CB L2-4/RConn2
  Three-Phase Breaker5/LConn3 -- Three-Phase Breaker6/LConn3 -- Three-Phase Breaker10/LConn3 -- Three-Phase Breaker9/LConn3 -- CB 25-beban/RConn3 -- Cap Bank RT2/LConn3 -- Three-Phase Breaker8/LConn3 -- Three-Phase Breaker7/LConn3
  CB 25-beban/LConn3 -- Trafo 2 SD 70:20/RConn3
  Three-Phase Breaker5/LConn1 -- Three-Phase Breaker6/LConn1 -- CB 25-beban/RConn1 -- Cap Bank RT2/LConn1 -- Three-Phase Breaker10/LConn1 -- Three-Phase Breaker9/LConn1 -- Three-Phase Breaker8/LConn1 -- Three-Phase Breaker7/LConn1
  CB 25-beban/LConn2 -- Trafo 2 SD 70:20/RConn2
  Three-Phase Breaker6/RConn2 -- Industri sedang/LConn2
  CB L2-4/RConn3 -- Trafo 2 SD 70:20/LConn3 -- CB L2-3/RConn3 -- CB L2-1/LConn3 -- CB 24-Gardu 2/RConn3
  Three-Phase Breaker5/RConn3 -- Industri kecil/LConn3
  Three-Phase Breaker18/RConn1 -- Pangkalan Militer/LConn1
  Three-Phase Breaker16/RConn1 -- Kantor Lembaga/LConn1
  Three-Phase Breaker14/RConn2 -- RS/LConn2
  Three-Phase Breaker17/RConn3 -- Istana Negara/LConn3
  Three-Phase Breaker15/RConn1 -- Pusat Server Data/LConn1
  CB L3-4/RConn3 -- Trafo 3 SD 70:20/LConn3 -- CB L3-2/LConn3 -- CB 34-Gardu 3/RConn3 -- CB L3-1/LConn3
  Three-Phase Breaker16/RConn3 -- Kantor Lembaga/LConn3
  Three-Phase Breaker14/RConn1 -- RS/LConn1
  Three-Phase Breaker15/RConn2 -- Pusat Server Data/LConn2
  CB 35-beban/LConn2 -- Trafo 3 SD 70:20/RConn2
  Three-Phase Breaker14/RConn3 -- RS/LConn3
  CB L3-1/LConn2 -- Trafo 3 SD 70:20/LConn2 -- CB L3-2/LConn2 -- CB L3-4/RConn2 -- CB 34-Gardu 3/RConn2
  Three-Phase Breaker16/RConn2 -- Kantor Lembaga/LConn2
  Three-Phase Breaker14/LConn2 -- Three-Phase Breaker16/LConn2 -- Three-Phase Breaker18/LConn2 -- Cap Bank RT3/LConn2 -- CB 35-beban/RConn2 -- Three-Phase Breaker17/LConn2 -- Three-Phase Breaker15/LConn2
  CB L3-1/LConn1 -- Trafo 3 SD 70:20/LConn1 -- CB L3-2/LConn1 -- CB L3-4/RConn1 -- CB 34-Gardu 3/RConn1
  Three-Phase Breaker17/RConn1 -- Istana Negara/LConn1
  Three-Phase Breaker15/RConn3 -- Pusat Server Data/LConn3
  Three-Phase Breaker14/LConn1 -- Three-Phase Breaker15/LConn1 -- Three-Phase Breaker16/LConn1 -- Three-Phase Breaker18/LConn1 -- Cap Bank RT3/LConn1 -- CB 35-beban/RConn1 -- Three-Phase Breaker17/LConn1
  Three-Phase Breaker18/RConn2 -- Pangkalan Militer/LConn2
  CB 35-beban/LConn3 -- Trafo 3 SD 70:20/RConn3
  Three-Phase Breaker18/RConn3 -- Pangkalan Militer/LConn3
  Three-Phase Breaker17/RConn2 -- Istana Negara/LConn2
  CB 35-beban/LConn1 -- Trafo 3 SD 70:20/RConn1
  Three-Phase Breaker18/LConn3 -- Three-Phase Breaker17/LConn3 -- Three-Phase Breaker16/LConn3 -- Three-Phase Breaker15/LConn3 -- Three-Phase Breaker14/LConn3 -- Cap Bank RT3/LConn3 -- CB 35-beban/RConn3
  CB 46-47/RConn2 -- Cap Bank RT4/LConn2 -- Trafo 5 SD 20:0.38/LConn2
  Three-Phase Breaker12/RConn1 -- Univ - Sekolah/LConn1
  Three-Phase Breaker13/RConn2 -- Rumah ibadah/LConn2
  Three-Phase Breaker11/RConn3 -- Penerangan Jalan/LConn3
  Three-Phase Breaker11/RConn2 -- Penerangan Jalan/LConn2
  Three-Phase Breaker11/RConn1 -- Penerangan Jalan/LConn1
  Three-Phase Breaker12/RConn3 -- Univ - Sekolah/LConn3
  Three-Phase Breaker12/RConn2 -- Univ - Sekolah/LConn2
  Three-Phase Breaker13/RConn3 -- Rumah ibadah/LConn3
  Three-Phase Breaker33/LConn2 -- Three-Phase Breaker34/LConn2 -- Three-Phase Breaker31/LConn2 -- Three-Phase Breaker13/LConn2 -- CB 47-beban/RConn2 -- Three-Phase Breaker12/LConn2 -- Three-Phase Breaker11/LConn2 -- Three-Phase Breaker30/LConn2 -- Three-Phase Breaker29/LConn2 -- Three-Phase Breaker32/LConn2
  Three-Phase Breaker13/RConn1 -- Rumah ibadah/LConn1
  CB 46-47/RConn1 -- Cap Bank RT4/LConn1 -- Trafo 5 SD 20:0.38/LConn1
  CB 46-47/RConn3 -- Trafo 5 SD 20:0.38/LConn3 -- Cap Bank RT4/LConn3
  Three-Phase Breaker33/LConn1 -- Three-Phase Breaker32/LConn1 -- Three-Phase Breaker34/LConn1 -- Three-Phase Breaker31/LConn1 -- Three-Phase Breaker13/LConn1 -- CB 47-beban/RConn1 -- Three-Phase Breaker12/LConn1 -- Three-Phase Breaker11/LConn1 -- Three-Phase Breaker30/LConn1 -- Three-Phase Breaker29/LConn1
  Three-Phase Breaker32/LConn3 -- Three-Phase Breaker33/LConn3 -- Three-Phase Breaker30/LConn3 -- Three-Phase Breaker31/LConn3 -- Three-Phase Breaker12/LConn3 -- Three-Phase Breaker13/LConn3 -- CB 47-beban/RConn3 -- Three-Phase Breaker11/LConn3 -- Three-Phase Breaker29/LConn3 -- Three-Phase Breaker34/LConn3
  CB 47-beban/LConn3 -- Trafo 5 SD 20:0.38/RConn3
  CB 47-beban/LConn2 -- Trafo 5 SD 20:0.38/RConn2
  CB 47-beban/LConn1 -- Trafo 5 SD 20:0.38/RConn1
  CB 45-46/RConn2 -- CB 46-45/LConn2
  CB 45-46/RConn3 -- CB 46-45/LConn3
  Line beban 8/RConn3 -- CB 46-47/LConn3 -- Line beban 7/RConn3 -- Line beban 4/RConn3 -- Line beban 12/RConn3 -- Line beban 11/RConn3 -- Line beban 10/RConn3 -- Line beban 9/RConn3
  Line beban 10/LConn2 -- Line beban 12/LConn2 -- Line beban 11/LConn2 -- Line beban 9/LConn2 -- CB 46-45/RConn2 -- Line beban 8/LConn2 -- Line beban 7/LConn2 -- Line beban 4/LConn2
  Line beban 8/RConn1 -- CB 46-47/LConn1 -- Line beban 12/RConn1 -- Line beban 11/RConn1 -- Line beban 10/RConn1 -- Line beban 9/RConn1 -- Line beban 4/RConn1 -- Line beban 7/RConn1
  Line beban 9/LConn1 -- Line beban 12/LConn1 -- Line beban 11/LConn1 -- Line beban 10/LConn1 -- CB 46-45/RConn1 -- Line beban 7/LConn1 -- Line beban 4/LConn1 -- Line beban 8/LConn1
  Line beban 9/RConn2 -- Line beban 12/RConn2 -- Line beban 11/RConn2 -- Line beban 10/RConn2 -- CB 46-47/LConn2 -- Line beban 4/RConn2 -- Line beban 7/RConn2 -- Line beban 8/RConn2
  CB 45-46/RConn1 -- CB 46-45/LConn1
  Line beban 9/LConn3 -- Line beban 12/LConn3 -- Line beban 11/LConn3 -- Line beban 10/LConn3 -- Line beban 8/LConn3 -- CB 46-45/RConn3 -- Line beban 7/LConn3 -- Line beban 4/LConn3
  Trafo 1 SU 70:230/RConn2 -- CB 13-12/LConn2
  Line PLTP-Gardu 1/LConn3 -- Line PLTP-Gardu 2/LConn3 -- CB 13-12/RConn3
  Line PLTP-Gardu 1/LConn2 -- Line PLTP-Gardu 2/LConn2 -- CB 13-12/RConn2
  CB 13-14/LConn2 -- Line PLTP-Gardu 1/RConn2 -- Line PLTP-Gardu 2/RConn2
  Line PLTP-Gardu 2/RConn1 -- CB 13-14/LConn1 -- Line PLTP-Gardu 1/RConn1
  Line PLTP-Gardu 1/LConn1 -- Line PLTP-Gardu 2/LConn1 -- CB 13-12/RConn1
  Trafo 1 SU 70:230/RConn3 -- CB 13-12/LConn3
  Line PLTP-Gardu 2/RConn3 -- CB 13-14/LConn3 -- Line PLTP-Gardu 1/RConn3
  Trafo 1 SU 70:230/RConn1 -- CB 13-12/LConn1
  Trafo 2 SU 230:70/LConn1 -- CB 23-24/RConn1
  Trafo 2 SU 70:230/RConn3 -- CB 23-22/LConn3
  Trafo 2 SU 230:70/LConn3 -- CB 23-24/RConn3
  Trafo 2 SU 70:230/RConn1 -- CB 23-22/LConn1
  CB 23-22/RConn1 -- Line PLTU-Gardu 1/LConn1 -- Line PLTU-Gardu 2/LConn1
  CB 23-22/RConn2 -- Line PLTU-Gardu 1/LConn2 -- Line PLTU-Gardu 2/LConn2
  Line PLTU-Gardu 2/RConn2 -- Line PLTU-Gardu 1/RConn2 -- CB 23-24/LConn2
  Line PLTU-Gardu 2/RConn1 -- Line PLTU-Gardu 1/RConn1 -- CB 23-24/LConn1
  Line PLTU-Gardu 2/RConn3 -- Line PLTU-Gardu 1/RConn3 -- CB 23-24/LConn3
  CB 23-22/RConn3 -- Line PLTU-Gardu 1/LConn3 -- Line PLTU-Gardu 2/LConn3
  Trafo 3 SU 230:70/LConn1 -- CB 33-34/RConn1
  Trafo 3 SU 230:70/LConn2 -- CB 33-34/RConn2
  Trafo 3 SU 70:230/RConn3 -- CB 33-32/LConn3
  Trafo 3 SU 230:70/LConn3 -- CB 33-34/RConn3
  Trafo 3 SU 70:230/RConn2 -- CB 33-32/LConn2
  "Line PLTA-Gardu 3 "/RConn3 -- Line PLTA-Gardu 3 1/RConn3 -- CB 33-34/LConn3
  Trafo 3 SU 70:230/RConn1 -- CB 33-32/LConn1
  "Line PLTA-Gardu 3 "/RConn2 -- Line PLTA-Gardu 3 1/RConn2 -- CB 33-34/LConn2
  CB 33-32/RConn1 -- Line PLTA-Gardu 3 1/LConn1 -- "Line PLTA-Gardu 3 "/LConn1
  CB 33-32/RConn2 -- Line PLTA-Gardu 3 1/LConn2 -- "Line PLTA-Gardu 3 "/LConn2
  CB 33-32/RConn3 -- Line PLTA-Gardu 3 1/LConn3 -- "Line PLTA-Gardu 3 "/LConn3
  "Line PLTA-Gardu 3 "/RConn1 -- Line PLTA-Gardu 3 1/RConn1 -- CB 33-34/LConn1
  Trafo 4 SU 70:1/RConn3 -- CB 43-42/LConn3
  Trafo 4 SU 70:1/RConn2 -- CB 43-42/LConn2
  CB 43-42/RConn1 -- Line PLTB-Gardu  1/LConn1 -- Line PLTB-Gardu  4/LConn1
  Line PLTB-Gardu  4/RConn2 -- Line PLTB-Gardu  1/RConn2 -- CB 43-44/LConn2
  Line PLTB-Gardu  4/RConn1 -- Line PLTB-Gardu  1/RConn1 -- CB 43-44/LConn1
  CB 43-42/RConn2 -- Line PLTB-Gardu  1/LConn2 -- Line PLTB-Gardu  4/LConn2
  Trafo 4 SU 70:1/RConn1 -- CB 43-42/LConn1
  Line PLTB-Gardu  4/RConn3 -- Line PLTB-Gardu  1/RConn3 -- CB 43-44/LConn3
  CB 43-42/RConn3 -- Line PLTB-Gardu  1/LConn3 -- Line PLTB-Gardu  4/LConn3
  Three-Phase Breaker23/RConn3 -- RT5.2/LConn3
  Three-Phase Breaker23/RConn1 -- RT5.2/LConn1
  Three-Phase Breaker23/RConn2 -- RT5.2/LConn2
  Three-Phase Breaker21/RConn2 -- RT3.2/LConn2
  Three-Phase Breaker20/RConn3 -- RT2.2/LConn3
  Three-Phase Breaker20/RConn2 -- RT2.2/LConn2
  Three-Phase Breaker19/RConn3 -- RT1.2/LConn3
  Three-Phase Breaker20/RConn1 -- RT2.2/LConn1
  Three-Phase Breaker21/RConn3 -- RT3.2/LConn3
  Three-Phase Breaker19/RConn2 -- RT1.2/LConn2
  Three-Phase Breaker22/RConn3 -- RT4.2/LConn3
  Three-Phase Breaker21/RConn1 -- RT3.2/LConn1
  Three-Phase Breaker22/RConn1 -- RT4.2/LConn1
  Three-Phase Breaker22/RConn2 -- RT4.2/LConn2
  Three-Phase Breaker19/RConn1 -- RT1.2/LConn1
  Three-Phase Breaker27/RConn3 -- RT4.3/LConn3
  Three-Phase Breaker28/RConn1 -- RT5.3/LConn1
  Three-Phase Breaker28/RConn3 -- RT5.3/LConn3
  Three-Phase Breaker24/RConn2 -- RT1.3/LConn2
  Three-Phase Breaker25/RConn1 -- RT2.3/LConn1
  Three-Phase Breaker27/RConn2 -- RT4.3/LConn2
  Three-Phase Breaker27/RConn1 -- RT4.3/LConn1
  Three-Phase Breaker25/RConn2 -- RT2.3/LConn2
  Three-Phase Breaker26/RConn3 -- RT3.3/LConn3
  Three-Phase Breaker28/RConn2 -- RT5.3/LConn2
  Three-Phase Breaker25/RConn3 -- RT2.3/LConn3
  Three-Phase Breaker26/RConn1 -- RT3.3/LConn1
  Three-Phase Breaker24/RConn1 -- RT1.3/LConn1
  Three-Phase Breaker24/RConn3 -- RT1.3/LConn3
  Three-Phase Breaker26/RConn2 -- RT3.3/LConn2
  Three-Phase Breaker31/RConn2 -- Rumah Ibadah 2/LConn2
  Three-Phase Breaker31/RConn3 -- Rumah Ibadah 2/LConn3
  Three-Phase Breaker30/RConn1 -- Univ - Sekolah 2/LConn1
  Three-Phase Breaker31/RConn1 -- Rumah Ibadah 2/LConn1
  Three-Phase Breaker29/RConn2 -- Penerangan Jalan 2/LConn2
  Three-Phase Breaker30/RConn3 -- Univ - Sekolah 2/LConn3
  Three-Phase Breaker29/RConn3 -- Penerangan Jalan 2/LConn3
  Three-Phase Breaker29/RConn1 -- Penerangan Jalan 2/LConn1
  Three-Phase Breaker30/RConn2 -- Univ - Sekolah 2/LConn2
  Three-Phase Breaker32/RConn1 -- Penerangan Jalan 3/LConn1
  Three-Phase Breaker32/RConn3 -- Penerangan Jalan 3/LConn3
  Three-Phase Breaker33/RConn1 -- Univ - Sekolah 3/LConn1
  Three-Phase Breaker32/RConn2 -- Penerangan Jalan 3/LConn2
  Three-Phase Breaker34/RConn1 -- Rumah Ibadah 3/LConn1
  Three-Phase Breaker33/RConn2 -- Univ - Sekolah 3/LConn2
  Three-Phase Breaker34/RConn2 -- Rumah Ibadah 3/LConn2
  Three-Phase Breaker34/RConn3 -- Rumah Ibadah 3/LConn3
  Three-Phase Breaker33/RConn3 -- Univ - Sekolah 3/LConn3
  Three-Phase Breaker21/LConn1 -- Three-Phase Breaker26/LConn1 -- Three-Phase Breaker24/LConn1 -- Three-Phase Breaker25/LConn1 -- Three-Phase Breaker27/LConn1 -- Three-Phase Breaker28/LConn1 -- Three-Phase Breaker19/LConn1 -- Three-Phase Breaker20/LConn1 -- Three-Phase Breaker4/LConn1 -- Three-Phase Breaker3/LConn1 -- Three-Phase Breaker2/LConn1 -- Three-Phase Breaker1/LConn1 -- Three-Phase Breaker/LConn1 -- Three-Phase Breaker23/LConn1 -- Three-Phase Breaker22/LConn1 -- CB 17-beban/RConn1
  CB 17-beban/RConn2 -- Three-Phase Breaker24/LConn2 -- Three-Phase Breaker25/LConn2 -- Three-Phase Breaker26/LConn2 -- Three-Phase Breaker27/LConn2 -- Three-Phase Breaker28/LConn2 -- Three-Phase Breaker19/LConn2 -- Three-Phase Breaker20/LConn2 -- Three-Phase Breaker21/LConn2 -- Three-Phase Breaker4/LConn2 -- Three-Phase Breaker3/LConn2 -- Three-Phase Breaker2/LConn2 -- Three-Phase Breaker1/LConn2 -- Three-Phase Breaker23/LConn2 -- Three-Phase Breaker/LConn2 -- Three-Phase Breaker22/LConn2
  CB 17-beban/RConn3 -- Three-Phase Breaker24/LConn3 -- Three-Phase Breaker25/LConn3 -- Three-Phase Breaker26/LConn3 -- Three-Phase Breaker27/LConn3 -- Three-Phase Breaker28/LConn3 -- Three-Phase Breaker19/LConn3 -- Three-Phase Breaker20/LConn3 -- Three-Phase Breaker21/LConn3 -- Three-Phase Breaker4/LConn3 -- Three-Phase Breaker3/LConn3 -- Three-Phase Breaker2/LConn3 -- Three-Phase Breaker1/LConn3 -- Three-Phase Breaker/LConn3 -- Three-Phase Breaker23/LConn3 -- Three-Phase Breaker22/LConn3
